simulink model "model_5LinkWalking"  (R2022b)
settings: Solver=ode45  StartTime=0.0  StopTime=Tf  FixedStep=1e-5  MaxStep=1e-3  RelTol=1e-12  AbsTol=1e-8
values from neighbouring files (symbols this model uses):
  f_dist = [0; -100; 0]    [main.m]    (also in main_5linkWalking_PSO.m)
  gains = [ ... (first row only)    [main.m]    (also in main_5linkWalking_PSO.m = [gain.kP1, gain.kD1, gain.kP2, gain.kD2, gain.kP3, gain.kD3,)
  gains_VSLIPSL = [gain_VSLIPSL.K_p; gain_VSLIPSL.K_d; gain_VSLIPSL.K_p_sw; gain_VSLIPSL.K_d_sw; gain_VSLIPSL.K_p_ds; gain_VSLIPSL.K_d_ds; gain_VSLIPSL.K_v_ds]    [main.m]    (also in main_5linkWalking_PSO.m)
  init_flag = [1; 0; -dc.col_param.footPlus; -slipsl.time_ss(N); slipsl.x_ss(1); slipsl.y_ss(1); alpha_ss_ref(1)]    [main.m]    (also in main_5linkWalking_PSO.m = [1; 0; -dc.col_param.footPlus; 0; CoM(1); CoM(2)])
  Initial_state = [q0;dq0]    [main.m]    (also in main_5linkWalking_PSO.m)
  param = [params.m1; params.m2; params.m5; params.l1; params.l2; params.l5; params.g; params.I1; params.I2; params.I5; params.r_k; params.r_h; params.k_ba; params.phi_h0; params.phi_k0]    [main.m]    (also in main_5linkWalking_PSO.m = [params.m1; params.m2; params.m5; params.l1; params.l2; para)
  ref_star_ds = [ref_star.ds.x_CoM_star,      ref_star.ds.y_CoM_star, ref_star.ds.dx_CoM_star,      ref_star.ds.del_y_CoM_star, ref_star.ds.del_dx_CoM_star,      ref_star.ds.del2_y_CoM_star]    [main.m]    (also in main_5linkWalking_PSO.m)
  ref_star_ss = [ref_star.ss.x_M_star,      ref_star.ss.y_M_star, ref_star.ss.x_swFoot_star, ref_star.ss.y_swFoot_star,      ref_star.ss.del_y_M_star, ref_star.ss.del_x_swFoot_star, ref_star.ss.del_y_swFoot_star,      ref_star.ss.del2_y_M_star, ref_star.ss.del2_x_swFoot_star, ref_star.ss.del2_y_swFoot_star,      ref_star.ss.x_CoM_star]    [main.m]    (also in main_5linkWalking_PSO.m)
  sample_time = 0.001    [main.m]    (also in main_5linkWalking_PSO.m)
  slipslParams = [ ... (first row only)    [main.m]    (also in main_5linkWalking_PSO.m)
  slipslTraj_ds = [slipsl.time_ds, slipsl.x_ds, slipsl.y_ds, slipsl.dx_ds, slipsl.dy_ds, alpha_ds_ref_discrete]    [main.m]    (also in main_5linkWalking_PSO.m = [ref_star.dc.ds.time - ref_star.dc.ds.time(1), ref_star.dc.d)
  slipslTraj_ss = [slipsl.time_ss, slipsl.x_ss, slipsl.y_ss, slipsl.dx_ss, slipsl.dy_ss, alpha_ss_ref_discrete]    [main.m]    (also in main_5linkWalking_PSO.m = [ref_star.dc.ss.time, ref_star.dc.ss.x_CoM', ref_star.dc.ss.)
  swFootTraj = [swFootSLIPSL.x_CoM, swFootSLIPSL.x, swFootSLIPSL.z, swFootSLIPSL.dx, swFootSLIPSL.dz]    [main.m]    (also in main_5linkWalking_PSO.m = [ref_star.dc.ss.x_CoM', ref_star.dc.ss.x_sw', ref_star.dc.ss)
libraries: simulink x1
(part 2 of 3)

== matlab function model_5LinkWalking/SLIP-SL Controller/SLIP-SL ==
  data: t input; des_traj output; X input; param input; flag input; slipslParams input; slipslTraj_ss input; slipslTraj_ds input; flag_des output; swFootTraj input; gains_VSLIPSL input; ref_star_ss input; ref_star_ds input; input_varStiff output; det_A_ds output; sw_ft_des output; des_th output; decoder_time_elapsed output; encoder_time_elapsed output
function [des_traj, flag_des, input_varStiff, det_A_ds, sw_ft_des, des_th, decoder_time_elapsed, encoder_time_elapsed] = fcn(t, X, param, flag, slipslParams, slipslTraj_ss, slipslTraj_ds, swFootTraj, gains_VSLIPSL, ref_star_ss, ref_star_ds)

%% variables (absolute angles)
th1 = X(1);
th2 = X(1) + X(2);
th3 = X(1) + X(2) + X(3);
th4 = X(1) + X(2) + X(3) + X(4);
th5 = X(1) + X(2) + X(5);

dth1 = X(6);
dth2 = X(6) + X(7);
dth3 = X(6) + X(7) + X(8);
dth4 = X(6) + X(7) + X(8) + X(9);
dth5 = X(6) + X(7) + X(10);

q = [th1;th2;th3;th4;th5];
dq = [dth1;dth2;dth3;dth4;dth5];

%% Parameters

m1 = param(1);
m2 = param(2);
m3 = m2;
m4 = m1;
m5 = param(3);

l1 = param(4);
l2 = param(5);
l5 = param(6);
l3 = l2;
l4 = l1;

gravi = param(7);
I1 = param(8);
I2 = param(9);
I5 = param(10);
I3 = I1;
I4 = I2;

%% flags
f_SS = flag(1); % indicates which stance phase it is
foot = flag(2); % location of the stance foot
foot_prev = flag(3); % previous location of the stance foot

t_mode_change = flag(4); % time stamp when the mode change happens (TD or LO)

x_LO = flag(5); % lift off location of CoM when it happened

%% CoM desired position and velocity calculation

time_ss = slipslTraj_ss(:,1);
x_slip_ss = slipslTraj_ss(:,2);
y_slip_ss = slipslTraj_ss(:,3);
dx_slip_ss = slipslTraj_ss(:,4);
dy_slip_ss = slipslTraj_ss(:,5);

time_ds = slipslTraj_ds(:,1);
x_slip_ds = slipslTraj_ds(:,2);
y_slip_ds = slipslTraj_ds(:,3);
dx_slip_ds = slipslTraj_ds(:,4);
dy_slip_ds = slipslTraj_ds(:,5);

CoM = calculate_com(X, param, foot, [0;0;0;0;0]); % calculating the location of CoM

x_CoM = CoM(1);
% z_CoM = CoM(2);
% dx_CoM = CoM(3); % velocity of CoM in x dir
% dz_CoM = CoM(4); % velocity of CoM in z dir

t_curr_step = t - t_mode_change; % timer for the current step, relative to the LO or TD time

if f_SS == 1
    % if we are in the SS phase
    
    if t_curr_step <= time_ss(end)
        % if the current time is within the SLIP-SL SS time
        
        x_CoM_des = interp1(time_ss, x_slip_ss, t_curr_step) + foot;
        y_CoM_des = interp1(time_ss, y_slip_ss, t_curr_step);
        dx_CoM_des = interp1(time_ss, dx_slip_ss, t_curr_step);
        dy_CoM_des = interp1(time_ss, dy_slip_ss, t_curr_step);
        
        flag_des = 1; % desired stance of the robot according to the slip traj
    else
        % if the current time has passed the time defined in SLIP-SL traj
        % (i.e. transition to DS is late)
        
%         x_CoM_des = x_slip_ss(end) + foot;
%         y_CoM_des = y_slip_ss(end);
%         dx_CoM_des = dx_slip_ss(end);
%         dy_CoM_des = dy_slip_ss(end);
        
        x_CoM_des = x_CoM; % current position of the x_CoM
        y_CoM_des = y_slip_ss(end);
        dx_CoM_des = dx_slip_ss(end);
        dy_CoM_des = dy_slip_ss(end);
        
        flag_des = 2; % desired stance of the robot according to the slip traj
    end
    
else
    % if we are in the DS phase
    
    footPlus = slipslParams(17); % position of footPlus for reference traj
    
    if t_curr_step <= time_ds(end)
        % if the current time is within the SLIP-SL DS time
        
        x_CoM_des = interp1(time_ds, x_slip_ds, t_curr_step) + foot - footPlus;
        y_CoM_des = interp1(time_ds, y_slip_ds, t_curr_step);
        dx_CoM_des = interp1(time_ds, dx_slip_ds, t_curr_step);
        dy_CoM_des = interp1(time_ds, dy_slip_ds, t_curr_step);
        
        flag_des = 2; % desired stance of the robot according to the slip traj
    else
        % if the current time has passed the time defined in SLIP-SL traj
        % (i.e. transition to SS is late)

        x_CoM_des = x_slip_ds(end) + foot - footPlus;
        y_CoM_des = y_slip_ds(end);
        dx_CoM_des = dx_slip_ds(end);
        dy_CoM_des = dy_slip_ds(end);
        
        flag_des = 1; % desired stance of the robot according to the slip traj
    end
end

%% SW foot desired position and velocity calculation

if f_SS == 1
    
    if t_curr_step <= time_ss(end)
        % if the x_CoM is within known SLIP-SL bounds
        x_sw_des = interp1(time_ss, swFootTraj(:,2) + foot, t_curr_step);
        y_sw_des = interp1(time_ss, swFootTraj(:,3), t_curr_step);
        dx_sw_des = interp1(time_ss, swFootTraj(:,4), t_curr_step);
        dy_sw_des = interp1(time_ss, swFootTraj(:,5), t_curr_step);
    else
        % if x_CoM goes out of SLIP-SL bounds, just use the last know ref. traj
        x_sw_des = swFootTraj(end,2) + foot;
        y_sw_des = swFootTraj(end,3);
        dx_sw_des = swFootTraj(end,4);
        % dy_sw_des = swFootTraj(end,5);
        dy_sw_des = swFootTraj(end,5) - 0.5*(t_curr_step - time_ss(end));
    end
    
else
    x_sw_des = foot_prev;
    y_sw_des = 0;
    dx_sw_des = 0;
    dy_sw_des = 0;
    
end

sw_ft_des = [x_sw_des; y_sw_des; dx_sw_des; dy_sw_des];

%% Desired accelerations calculation

% SLIP-SL constant params
m_M = slipslParams(1);
m_swLeg = slipslParams(2);
m_swFoot = slipslParams(3);
L_thigh = slipslParams(4);
I_swLeg = slipslParams(5);
I_swFoot = slipslParams(6);
gravi = slipslParams(7);

% SLIP-SL collocation parameters
k0_ss = slipslParams(8);
L0_ss = slipslParams(9);
k0_ds = slipslParams(10);
L0_ds = slipslParams(11);
k_swFoot = slipslParams(12);
k_swLeg = slipslParams(13);
theta0 = slipslParams(14);
r0 = slipslParams(15);
foot = slipslParams(16);
footPlus = slipslParams(17);

%%%%% V-SLIP-SL controller that calculates variable stiffness inputs %%%%%

% SS inputs
u1 = 0; % input for stance leg spring
u2 = 0; % input for swing leg torsional spring
u3 = 0; % input for swing foot spring
% DS inputs
u4 = 0; % input for stance leg spring
u5 = 0; % input for swing leg spring

% Controller Gains
K_p = gains_VSLIPSL(1);
K_d = gains_VSLIPSL(2);

K_p_sw = gains_VSLIPSL(3);
K_d_sw = gains_VSLIPSL(4);

K_p_ds = gains_VSLIPSL(5);
K_d_ds = gains_VSLIPSL(6);
K_v_ds = gains_VSLIPSL(7); % 5 in visser 2012

% for debugging
ref_output_ss = [0; 0; 0];
ref_output_ds = [0;0];
det_A_ss = -1;
det_A_ds = 0;

x_CoM_star_ds = ref_star_ds(:,1);
%%%%%%%%%%%%%%%%%%%%%%%%%%%%%%%%%%%%%%%%%%%%%%%%%%%%%%%%%%%%%%%%%%%%%%%%%%

encoder_time_elapsed = NaN;

if f_SS == 1
    % if the 5 link model is in SS
    
    if t_curr_step <= time_ss(end)
        % (SS) SLIP-SL states corresponding to current x_CoM position
        
        [x_M, y_M, theta, r, dx_M, dy_M, dtheta, dr, encoder_time_elapsed] = calc_5linkTOslipsl(X, flag, param, slipslParams);
        
        %%%%%% V-SLIP-SL SS Phase Controller %%%%%%%%%%%%%%%%%%%%%%%%%%%%%
        x_CoM_star_ss = ref_star_ss(:,11);
        x_M_star_ss = ref_star_ss(:,1);
        x_swFoot_ref = ref_star_ss(:,3);
        
        % updating the x_CoM_star_ss
        x_CoM_des_TD = ref_star_ss(end,11);
        x_CoM_star_ss = x_CoM_star_ss.*((x_CoM_des_TD - (x_LO-flag(2)))/(ref_star_ss(end,11) - ref_star_ss(1,11))) + ((x_LO-flag(2)) - ref_star_ss(1,11))/2;
        
        % calculating x_CoM when for SS phase
        x_swLeg = x_M + (L_thigh/2)*cos(theta);
        x_swFoot = x_M + (L_thigh + r)*cos(theta);
%         x_CoM = (m_M*x_M + m_swLeg*x_swLeg + m_swFoot*x_swFoot)/(m_M + m_swLeg + m_swFoot);
        x_CoM = CoM(1) - flag(2);
        
        if x_CoM_star_ss(1) <= x_CoM && x_CoM <= x_CoM_star_ss(end)
            %
            %     if x_M <= x_M_star_ss(end)
            
            % interpolation for references
            y_M_star = interp1(x_CoM_star_ss, ref_star_ss(:,2), x_CoM);
            %         x_swFoot_star = interp1(x_M_star_ss, x_swFoot_ref_mod, x_M);
            x_swFoot_star = interp1(x_CoM_star_ss, ref_star_ss(:,3), x_CoM);
            y_swFoot_star = interp1(x_CoM_star_ss, ref_star_ss(:,4), x_CoM);
            
            del_y_M_star = interp1(x_CoM_star_ss, ref_star_ss(:,5), x_CoM);
            del_x_swFoot_star = interp1(x_CoM_star_ss, ref_star_ss(:,6), x_CoM);
            del_y_swFoot_star = interp1(x_CoM_star_ss, ref_star_ss(:,7), x_CoM);
            
            del2_y_M_star = interp1(x_CoM_star_ss, ref_star_ss(:,8), x_CoM);
            del2_x_swFoot_star = interp1(x_CoM_star_ss, ref_star_ss(:,9), x_CoM);
            del2_y_swFoot_star = interp1(x_CoM_star_ss, ref_star_ss(:,10), x_CoM);

%             % interpolation for references (trying time based instead of x_CoM based
%             y_M_star = interp1(x_CoM_star_ss, ref_star_ss(:,2), x_CoM);
%             %         x_swFoot_star = interp1(x_M_star_ss, x_swFoot_ref_mod, x_M);
%             x_swFoot_star = interp1(x_CoM_star_ss, ref_star_ss(:,3), x_CoM);
%             y_swFoot_star = interp1(x_CoM_star_ss, ref_star_ss(:,4), x_CoM);
%             
%             del_y_M_star = interp1(x_CoM_star_ss, ref_star_ss(:,5), x_CoM);
%             del_x_swFoot_star = interp1(x_CoM_star_ss, ref_star_ss(:,6), x_CoM);
%             del_y_swFoot_star = interp1(x_CoM_star_ss, ref_star_ss(:,7), x_CoM);
%             
%             del2_y_M_star = interp1(x_CoM_star_ss, ref_star_ss(:,8), x_CoM);
%             del2_x_swFoot_star = interp1(x_CoM_star_ss, ref_star_ss(:,9), x_CoM);
%             del2_y_swFoot_star = interp1(x_CoM_star_ss, ref_star_ss(:,10), x_CoM);
            
            ref_output_ss = [y_M_star; x_swFoot_star; y_swFoot_star];
            
            % controller
            
            A_ss = [
                ((L0_ss - (x_M^2 + y_M^2)^(1/2))*(L_thigh^2*m_swLeg^2*y_M + 8*I_swLeg*m_M*y_M + 8*I_swFoot*m_M*y_M + 8*I_swLeg*m_swLeg*y_M + 4*I_swLeg*m_swFoot*y_M + 8*I_swFoot*m_swLeg*y_M + 4*I_swFoot*m_swFoot*y_M + 2*L_thigh^2*m_M*m_swLeg*y_M + 8*L_thigh^2*m_M*m_swFoot*y_M + 5*L_thigh^2*m_swLeg*m_swFoot*y_M + 8*m_M*m_swFoot*r^2*y_M + 8*m_swLeg*m_swFoot*r^2*y_M + L_thigh^2*m_swLeg^2*y_M*cos(2*theta) - L_thigh^2*m_swLeg^2*x_M*sin(2*theta) - 4*I_swLeg*m_swFoot*y_M*cos(2*theta) - 4*I_swFoot*m_swFoot*y_M*cos(2*theta) + 4*I_swLeg*m_swFoot*x_M*sin(2*theta) + 4*I_swFoot*m_swFoot*x_M*sin(2*theta) + 16*L_thigh*m_M*m_swFoot*r*y_M + 12*L_thigh*m_swLeg*m_swFoot*r*y_M + 3*L_thigh^2*m_swLeg*m_swFoot*y_M*cos(2*theta) - 3*L_thigh^2*m_swLeg*m_swFoot*x_M*sin(2*theta) + 4*L_thigh*m_swLeg*m_swFoot*r*y_M*cos(2*theta) - 4*L_thigh*m_swLeg*m_swFoot*r*x_M*sin(2*theta)))/(2*(x_M^2 + y_M^2)^(1/2)*(m_M + m_swLeg)*(4*I_swLeg*m_M + 4*I_swFoot*m_M + 4*I_swLeg*m_swLeg + 4*I_swLeg*m_swFoot + 4*I_swFoot*m_swLeg + 4*I_swFoot*m_swFoot + 4*m_M*m_swFoot*r^2 + 4*m_swLeg*m_swFoot*r^2 + L_thigh^2*m_M*m_swLeg + 4*L_thigh^2*m_M*m_swFoot + L_thigh^2*m_swLeg*m_swFoot + 8*L_thigh*m_M*m_swFoot*r + 4*L_thigh*m_swLeg*m_swFoot*r)) - (del_y_M_star*(L0_ss - (x_M^2 + y_M^2)^(1/2))*((L_thigh^2*m_swLeg^2*x_M)/2 + 4*I_swLeg*m_M*x_M + 4*I_swFoot*m_M*x_M + 4*I_swLeg*m_swLeg*x_M + 2*I_swLeg*m_swFoot*x_M + 4*I_swFoot*m_swLeg*x_M + 2*I_swFoot*m_swFoot*x_M + L_thigh^2*m_M*m_swLeg*x_M + 4*L_thigh^2*m_M*m_swFoot*x_M + (5*L_thigh^2*m_swLeg*m_swFoot*x_M)/2 + 4*m_M*m_swFoot*r^2*x_M + 4*m_swLeg*m_swFoot*r^2*x_M - (L_thigh^2*m_swLeg^2*x_M*cos(2*theta))/2 - (L_thigh^2*m_swLeg^2*y_M*sin(2*theta))/2 + 2*I_swLeg*m_swFoot*x_M*cos(2*theta) + 2*I_swFoot*m_swFoot*x_M*cos(2*theta) + 2*I_swLeg*m_swFoot*y_M*sin(2*theta) + 2*I_swFoot*m_swFoot*y_M*sin(2*theta) + 8*L_thigh*m_M*m_swFoot*r*x_M + 6*L_thigh*m_swLeg*m_swFoot*r*x_M - (3*L_thigh^2*m_swLeg*m_swFoot*x_M*cos(2*theta))/2 - (3*L_thigh^2*m_swLeg*m_swFoot*y_M*sin(2*theta))/2 - 2*L_thigh*m_swLeg*m_swFoot*r*x_M*cos(2*theta) - 2*L_thigh*m_swLeg*m_swFoot*r*y_M*sin(2*theta)))/((x_M^2 + y_M^2)^(1/2)*(m_M + m_swLeg)*(4*I_swLeg*m_M + 4*I_swFoot*m_M + 4*I_swLeg*m_swLeg + 4*I_swLeg*m_swFoot + 4*I_swFoot*m_swLeg + 4*I_swFoot*m_swFoot + 4*m_M*m_swFoot*r^2 + 4*m_swLeg*m_swFoot*r^2 + L_thigh^2*m_M*m_swLeg + 4*L_thigh^2*m_M*m_swFoot + L_thigh^2*m_swLeg*m_swFoot + 8*L_thigh*m_M*m_swFoot*r + 4*L_thigh*m_swLeg*m_swFoot*r)),                                                                                                                                                        (2*(theta - theta0)*(cos(theta) + del_y_M_star*sin(theta))*(L_thigh*m_swLeg + 2*L_thigh*m_swFoot + 2*m_swFoot*r))/(4*I_swLeg*m_M + 4*I_swFoot*m_M + 4*I_swLeg*m_swLeg + 4*I_swLeg*m_swFoot + 4*I_swFoot*m_swLeg + 4*I_swFoot*m_swFoot + 4*m_M*m_swFoot*r^2 + 4*m_swLeg*m_swFoot*r^2 + L_thigh^2*m_M*m_swLeg + 4*L_thigh^2*m_M*m_swFoot + L_thigh^2*m_swLeg*m_swFoot + 8*L_thigh*m_M*m_swFoot*r + 4*L_thigh*m_swLeg*m_swFoot*r),                                                    ((r - r0)*(sin(theta) - del_y_M_star*cos(theta)))/(m_M + m_swLeg)
                (2*sin(theta)*(L_thigh + r)*(L0_ss - (x_M^2 + y_M^2)^(1/2))*(y_M*cos(theta) - x_M*sin(theta))*(L_thigh*m_swLeg + 2*L_thigh*m_swFoot + 2*m_swFoot*r))/((x_M^2 + y_M^2)^(1/2)*(4*I_swLeg*m_M + 4*I_swFoot*m_M + 4*I_swLeg*m_swLeg + 4*I_swLeg*m_swFoot + 4*I_swFoot*m_swLeg + 4*I_swFoot*m_swFoot + 4*m_M*m_swFoot*r^2 + 4*m_swLeg*m_swFoot*r^2 + L_thigh^2*m_M*m_swLeg + 4*L_thigh^2*m_M*m_swFoot + L_thigh^2*m_swLeg*m_swFoot + 8*L_thigh*m_M*m_swFoot*r + 4*L_thigh*m_swLeg*m_swFoot*r)) - ((L0_ss - (x_M^2 + y_M^2)^(1/2))*(del_x_swFoot_star - 1)*((L_thigh^2*m_swLeg^2*x_M)/2 + 4*I_swLeg*m_M*x_M + 4*I_swFoot*m_M*x_M + 4*I_swLeg*m_swLeg*x_M + 2*I_swLeg*m_swFoot*x_M + 4*I_swFoot*m_swLeg*x_M + 2*I_swFoot*m_swFoot*x_M + L_thigh^2*m_M*m_swLeg*x_M + 4*L_thigh^2*m_M*m_swFoot*x_M + (5*L_thigh^2*m_swLeg*m_swFoot*x_M)/2 + 4*m_M*m_swFoot*r^2*x_M + 4*m_swLeg*m_swFoot*r^2*x_M - (L_thigh^2*m_swLeg^2*x_M*cos(2*theta))/2 - (L_thigh^2*m_swLeg^2*y_M*sin(2*theta))/2 + 2*I_swLeg*m_swFoot*x_M*cos(2*theta) + 2*I_swFoot*m_swFoot*x_M*cos(2*theta) + 2*I_swLeg*m_swFoot*y_M*sin(2*theta) + 2*I_swFoot*m_swFoot*y_M*sin(2*theta) + 8*L_thigh*m_M*m_swFoot*r*x_M + 6*L_thigh*m_swLeg*m_swFoot*r*x_M - (3*L_thigh^2*m_swLeg*m_swFoot*x_M*cos(2*theta))/2 - (3*L_thigh^2*m_swLeg*m_swFoot*y_M*sin(2*theta))/2 - 2*L_thigh*m_swLeg*m_swFoot*r*x_M*cos(2*theta) - 2*L_thigh*m_swLeg*m_swFoot*r*y_M*sin(2*theta)))/((x_M^2 + y_M^2)^(1/2)*(m_M + m_swLeg)*(4*I_swLeg*m_M + 4*I_swFoot*m_M + 4*I_swLeg*m_swLeg + 4*I_swLeg*m_swFoot + 4*I_swFoot*m_swLeg + 4*I_swFoot*m_swFoot + 4*m_M*m_swFoot*r^2 + 4*m_swLeg*m_swFoot*r^2 + L_thigh^2*m_M*m_swLeg + 4*L_thigh^2*m_M*m_swFoot + L_thigh^2*m_swLeg*m_swFoot + 8*L_thigh*m_M*m_swFoot*r + 4*L_thigh*m_swLeg*m_swFoot*r)) - (cos(theta)*(L0_ss - (x_M^2 + y_M^2)^(1/2))*(x_M*cos(theta) + y_M*sin(theta)))/((x_M^2 + y_M^2)^(1/2)*(m_M + m_swLeg)),                                                                    (2*sin(theta)*(theta - theta0)*(2*L_thigh*m_M + L_thigh*m_swLeg + 2*m_M*r + 2*m_swLeg*r + L_thigh*del_x_swFoot_star*m_swLeg + 2*L_thigh*del_x_swFoot_star*m_swFoot + 2*del_x_swFoot_star*m_swFoot*r))/(4*I_swLeg*m_M + 4*I_swFoot*m_M + 4*I_swLeg*m_swLeg + 4*I_swLeg*m_swFoot + 4*I_swFoot*m_swLeg + 4*I_swFoot*m_swFoot + 4*m_M*m_swFoot*r^2 + 4*m_swLeg*m_swFoot*r^2 + L_thigh^2*m_M*m_swLeg + 4*L_thigh^2*m_M*m_swFoot + L_thigh^2*m_swLeg*m_swFoot + 8*L_thigh*m_M*m_swFoot*r + 4*L_thigh*m_swLeg*m_swFoot*r),                       -(cos(theta)*(r - r0)*(m_M + m_swLeg + del_x_swFoot_star*m_swFoot))/(m_swFoot*(m_M + m_swLeg))
                ((L0_ss - (x_M^2 + y_M^2)^(1/2))*(L_thigh^2*m_swLeg^2*y_M + 8*I_swLeg*m_M*y_M + 8*I_swFoot*m_M*y_M + 8*I_swLeg*m_swLeg*y_M + 4*I_swLeg*m_swFoot*y_M + 8*I_swFoot*m_swLeg*y_M + 4*I_swFoot*m_swFoot*y_M + 2*L_thigh^2*m_M*m_swLeg*y_M + 8*L_thigh^2*m_M*m_swFoot*y_M + 5*L_thigh^2*m_swLeg*m_swFoot*y_M + 8*m_M*m_swFoot*r^2*y_M + 8*m_swLeg*m_swFoot*r^2*y_M + L_thigh^2*m_swLeg^2*y_M*cos(2*theta) - L_thigh^2*m_swLeg^2*x_M*sin(2*theta) - 4*I_swLeg*m_swFoot*y_M*cos(2*theta) - 4*I_swFoot*m_swFoot*y_M*cos(2*theta) + 4*I_swLeg*m_swFoot*x_M*sin(2*theta) + 4*I_swFoot*m_swFoot*x_M*sin(2*theta) + 16*L_thigh*m_M*m_swFoot*r*y_M + 12*L_thigh*m_swLeg*m_swFoot*r*y_M + 3*L_thigh^2*m_swLeg*m_swFoot*y_M*cos(2*theta) - 3*L_thigh^2*m_swLeg*m_swFoot*x_M*sin(2*theta) + 4*L_thigh*m_swLeg*m_swFoot*r*y_M*cos(2*theta) - 4*L_thigh*m_swLeg*m_swFoot*r*x_M*sin(2*theta)))/(2*(x_M^2 + y_M^2)^(1/2)*(m_M + m_swLeg)*(4*I_swLeg*m_M + 4*I_swFoot*m_M + 4*I_swLeg*m_swLeg + 4*I_swLeg*m_swFoot + 4*I_swFoot*m_swLeg + 4*I_swFoot*m_swFoot + 4*m_M*m_swFoot*r^2 + 4*m_swLeg*m_swFoot*r^2 + L_thigh^2*m_M*m_swLeg + 4*L_thigh^2*m_M*m_swFoot + L_thigh^2*m_swLeg*m_swFoot + 8*L_thigh*m_M*m_swFoot*r + 4*L_thigh*m_swLeg*m_swFoot*r)) - (sin(theta)*(L0_ss - (x_M^2 + y_M^2)^(1/2))*(x_M*cos(theta) + y_M*sin(theta)))/((x_M^2 + y_M^2)^(1/2)*(m_M + m_swLeg)) - (del_y_swFoot_star*(L0_ss - (x_M^2 + y_M^2)^(1/2))*((L_thigh^2*m_swLeg^2*x_M)/2 + 4*I_swLeg*m_M*x_M + 4*I_swFoot*m_M*x_M + 4*I_swLeg*m_swLeg*x_M + 2*I_swLeg*m_swFoot*x_M + 4*I_swFoot*m_swLeg*x_M + 2*I_swFoot*m_swFoot*x_M + L_thigh^2*m_M*m_swLeg*x_M + 4*L_thigh^2*m_M*m_swFoot*x_M + (5*L_thigh^2*m_swLeg*m_swFoot*x_M)/2 + 4*m_M*m_swFoot*r^2*x_M + 4*m_swLeg*m_swFoot*r^2*x_M - (L_thigh^2*m_swLeg^2*x_M*cos(2*theta))/2 - (L_thigh^2*m_swLeg^2*y_M*sin(2*theta))/2 + 2*I_swLeg*m_swFoot*x_M*cos(2*theta) + 2*I_swFoot*m_swFoot*x_M*cos(2*theta) + 2*I_swLeg*m_swFoot*y_M*sin(2*theta) + 2*I_swFoot*m_swFoot*y_M*sin(2*theta) + 8*L_thigh*m_M*m_swFoot*r*x_M + 6*L_thigh*m_swLeg*m_swFoot*r*x_M - (3*L_thigh^2*m_swLeg*m_swFoot*x_M*cos(2*theta))/2 - (3*L_thigh^2*m_swLeg*m_swFoot*y_M*sin(2*theta))/2 - 2*L_thigh*m_swLeg*m_swFoot*r*x_M*cos(2*theta) - 2*L_thigh*m_swLeg*m_swFoot*r*y_M*sin(2*theta)))/((x_M^2 + y_M^2)^(1/2)*(m_M + m_swLeg)*(4*I_swLeg*m_M + 4*I_swFoot*m_M + 4*I_swLeg*m_swLeg + 4*I_swLeg*m_swFoot + 4*I_swFoot*m_swLeg + 4*I_swFoot*m_swFoot + 4*m_M*m_swFoot*r^2 + 4*m_swLeg*m_swFoot*r^2 + L_thigh^2*m_M*m_swLeg + 4*L_thigh^2*m_M*m_swFoot + L_thigh^2*m_swLeg*m_swFoot + 8*L_thigh*m_M*m_swFoot*r + 4*L_thigh*m_swLeg*m_swFoot*r)) - (2*cos(theta)*(L_thigh + r)*(L0_ss - (x_M^2 + y_M^2)^(1/2))*(y_M*cos(theta) - x_M*sin(theta))*(L_thigh*m_swLeg + 2*L_thigh*m_swFoot + 2*m_swFoot*r))/((x_M^2 + y_M^2)^(1/2)*(4*I_swLeg*m_M + 4*I_swFoot*m_M + 4*I_swLeg*m_swLeg + 4*I_swLeg*m_swFoot + 4*I_swFoot*m_swLeg + 4*I_swFoot*m_swFoot + 4*m_M*m_swFoot*r^2 + 4*m_swLeg*m_swFoot*r^2 + L_thigh^2*m_M*m_swLeg + 4*L_thigh^2*m_M*m_swFoot + L_thigh^2*m_swLeg*m_swFoot + 8*L_thigh*m_M*m_swFoot*r + 4*L_thigh*m_swLeg*m_swFoot*r)), -(2*(theta - theta0)*(2*m_M*r*cos(theta) + 2*m_swLeg*r*cos(theta) + 2*L_thigh*m_M*cos(theta) + L_thigh*m_swLeg*cos(theta) - L_thigh*del_y_swFoot_star*m_swLeg*sin(theta) - 2*L_thigh*del_y_swFoot_star*m_swFoot*sin(theta) - 2*del_y_swFoot_star*m_swFoot*r*sin(theta)))/(4*I_swLeg*m_M + 4*I_swFoot*m_M + 4*I_swLeg*m_swLeg + 4*I_swLeg*m_swFoot + 4*I_swFoot*m_swLeg + 4*I_swFoot*m_swFoot + 4*m_M*m_swFoot*r^2 + 4*m_swLeg*m_swFoot*r^2 + L_thigh^2*m_M*m_swLeg + 4*L_thigh^2*m_M*m_swFoot + L_thigh^2*m_swLeg*m_swFoot + 8*L_thigh*m_M*m_swFoot*r + 4*L_thigh*m_swLeg*m_swFoot*r), -((r - r0)*(m_M*sin(theta) + m_swLeg*sin(theta) + del_y_swFoot_star*m_swFoot*cos(theta)))/(m_swFoot*(m_M + m_swLeg))];
            
            K_ss = [
                del2_y_M_star*dx_M^2 - K_p*(y_M - y_M_star) - K_d*(dy_M - del_y_M_star*dx_M) + (8*I_swLeg*gravi*m_M^2*(x_M^2 + y_M^2)^(1/2) + 8*I_swFoot*gravi*m_M^2*(x_M^2 + y_M^2)^(1/2) + 8*I_swLeg*gravi*m_swLeg^2*(x_M^2 + y_M^2)^(1/2) + 8*I_swFoot*gravi*m_swLeg^2*(x_M^2 + y_M^2)^(1/2) - L0_ss*L_thigh^2*k0_ss*m_swLeg^2*y_M + 2*L_thigh^2*gravi*m_M*m_swLeg^2*(x_M^2 + y_M^2)^(1/2) + 2*L_thigh^2*gravi*m_M^2*m_swLeg*(x_M^2 + y_M^2)^(1/2) + 8*L_thigh^2*gravi*m_M^2*m_swFoot*(x_M^2 + y_M^2)^(1/2) + 2*L_thigh^2*gravi*m_swLeg^2*m_swFoot*(x_M^2 + y_M^2)^(1/2) + L_thigh^2*k0_ss*m_swLeg^2*y_M*(x_M^2 + y_M^2)^(1/2) + 8*gravi*m_M^2*m_swFoot*r^2*(x_M^2 + y_M^2)^(1/2) + 8*gravi*m_swLeg^2*m_swFoot*r^2*(x_M^2 + y_M^2)^(1/2) - 8*I_swLeg*L0_ss*k0_ss*m_M*y_M - 8*I_swFoot*L0_ss*k0_ss*m_M*y_M - 8*I_swLeg*L0_ss*k0_ss*m_swLeg*y_M - 4*I_swLeg*L0_ss*k0_ss*m_swFoot*y_M - 8*I_swFoot*L0_ss*k0_ss*m_swLeg*y_M - 4*I_swFoot*L0_ss*k0_ss*m_swFoot*y_M + 16*I_swLeg*gravi*m_M*m_swLeg*(x_M^2 + y_M^2)^(1/2) + 8*I_swLeg*gravi*m_M*m_swFoot*(x_M^2 + y_M^2)^(1/2) + 16*I_swFoot*gravi*m_M*m_swLeg*(x_M^2 + y_M^2)^(1/2) + 8*I_swFoot*gravi*m_M*m_swFoot*(x_M^2 + y_M^2)^(1/2) + 8*I_swLeg*gravi*m_swLeg*m_swFoot*(x_M^2 + y_M^2)^(1/2) + 8*I_swFoot*gravi*m_swLeg*m_swFoot*(x_M^2 + y_M^2)^(1/2) + 8*I_swLeg*k0_ss*m_M*y_M*(x_M^2 + y_M^2)^(1/2) + 8*I_swFoot*k0_ss*m_M*y_M*(x_M^2 + y_M^2)^(1/2) + 8*I_swLeg*k0_ss*m_swLeg*y_M*(x_M^2 + y_M^2)^(1/2) + 4*I_swLeg*k0_ss*m_swFoot*y_M*(x_M^2 + y_M^2)^(1/2) + 8*I_swFoot*k0_ss*m_swLeg*y_M*(x_M^2 + y_M^2)^(1/2) + 4*I_swFoot*k0_ss*m_swFoot*y_M*(x_M^2 + y_M^2)^(1/2) - 2*L0_ss*L_thigh^2*k0_ss*m_M*m_swLeg*y_M - 8*L0_ss*L_thigh^2*k0_ss*m_M*m_swFoot*y_M - 5*L0_ss*L_thigh^2*k0_ss*m_swLeg*m_swFoot*y_M + 10*L_thigh^2*gravi*m_M*m_swLeg*m_swFoot*(x_M^2 + y_M^2)^(1/2) + 16*L_thigh*gravi*m_M^2*m_swFoot*r*(x_M^2 + y_M^2)^(1/2) + 8*L_thigh*gravi*m_swLeg^2*m_swFoot*r*(x_M^2 + y_M^2)^(1/2) + 2*L_thigh^2*k0_ss*m_M*m_swLeg*y_M*(x_M^2 + y_M^2)^(1/2) + 8*L_thigh^2*k0_ss*m_M*m_swFoot*y_M*(x_M^2 + y_M^2)^(1/2) + 5*L_thigh^2*k0_ss*m_swLeg*m_swFoot*y_M*(x_M^2 + y_M^2)^(1/2) - 8*L0_ss*k0_ss*m_M*m_swFoot*r^2*y_M - 8*L0_ss*k0_ss*m_swLeg*m_swFoot*r^2*y_M - L0_ss*L_thigh^2*k0_ss*m_swLeg^2*y_M*cos(2*theta) - 8*I_swLeg*k_swFoot*m_M*r*sin(theta)*(x_M^2 + y_M^2)^(1/2) + 8*I_swLeg*k_swFoot*m_M*r0*sin(theta)*(x_M^2 + y_M^2)^(1/2) - 8*I_swFoot*k_swFoot*m_M*r*sin(theta)*(x_M^2 + y_M^2)^(1/2) + 8*I_swFoot*k_swFoot*m_M*r0*sin(theta)*(x_M^2 + y_M^2)^(1/2) - 8*I_swLeg*k_swFoot*m_swLeg*r*sin(theta)*(x_M^2 + y_M^2)^(1/2) + 8*I_swLeg*k_swFoot*m_swLeg*r0*sin(theta)*(x_M^2 + y_M^2)^(1/2) - 8*I_swLeg*k_swFoot*m_swFoot*r*sin(theta)*(x_M^2 + y_M^2)^(1/2) + 8*I_swLeg*k_swFoot*m_swFoot*r0*sin(theta)*(x_M^2 + y_M^2)^(1/2) - 8*I_swFoot*k_swFoot*m_swLeg*r*sin(theta)*(x_M^2 + y_M^2)^(1/2) + 8*I_swFoot*k_swFoot*m_swLeg*r0*sin(theta)*(x_M^2 + y_M^2)^(1/2) - 8*I_swFoot*k_swFoot*m_swFoot*r*sin(theta)*(x_M^2 + y_M^2)^(1/2) + 8*I_swFoot*k_swFoot*m_swFoot*r0*sin(theta)*(x_M^2 + y_M^2)^(1/2) + L0_ss*L_thigh^2*k0_ss*m_swLeg^2*x_M*sin(2*theta) + 16*gravi*m_M*m_swLeg*m_swFoot*r^2*(x_M^2 + y_M^2)^(1/2) + 8*k0_ss*m_M*m_swFoot*r^2*y_M*(x_M^2 + y_M^2)^(1/2) + 8*k0_ss*m_swLeg*m_swFoot*r^2*y_M*(x_M^2 + y_M^2)^(1/2) - L_thigh^3*dtheta^2*m_M*m_swLeg^2*sin(theta)*(x_M^2 + y_M^2)^(1/2) - L_thigh^3*dtheta^2*m_swLeg^2*m_swFoot*sin(theta)*(x_M^2 + y_M^2)^(1/2) + L_thigh^2*k0_ss*m_swLeg^2*y_M*cos(2*theta)*(x_M^2 + y_M^2)^(1/2) - L_thigh^2*k0_ss*m_swLeg^2*x_M*sin(2*theta)*(x_M^2 + y_M^2)^(1/2) + 4*I_swLeg*L0_ss*k0_ss*m_swFoot*y_M*cos(2*theta) + 4*I_swFoot*L0_ss*k0_ss*m_swFoot*y_M*cos(2*theta) - 4*I_swLeg*L0_ss*k0_ss*m_swFoot*x_M*sin(2*theta) - 4*I_swFoot*L0_ss*k0_ss*m_swFoot*x_M*sin(2*theta) - 4*L_thigh*k_swLeg*m_swLeg^2*theta*cos(theta)*(x_M^2 + y_M^2)^(1/2) + 4*L_thigh*k_swLeg*m_swLeg^2*theta0*cos(theta)*(x_M^2 + y_M^2)^(1/2) - 4*I_swLeg*k0_ss*m_swFoot*y_M*cos(2*theta)*(x_M^2 + y_M^2)^(1/2) - 4*I_swFoot*k0_ss*m_swFoot*y_M*cos(2*theta)*(x_M^2 + y_M^2)^(1/2) + 4*I_swLeg*k0_ss*m_swFoot*x_M*sin(2*theta)*(x_M^2 + y_M^2)^(1/2) + 4*I_swFoot*k0_ss*m_swFoot*x_M*sin(2*theta)*(x_M^2 + y_M^2)^(1/2) - 8*k_swFoot*m_M*m_swFoot*r^3*sin(theta)*(x_M^2 + y_M^2)^(1/2) - 8*k_swFoot*m_swLeg*m_swFoot*r^3*sin(theta)*(x_M^2 + y_M^2)^(1/2) - 4*I_swLeg*L_thigh*dtheta^2*m_swLeg^2*sin(theta)*(x_M^2 + y_M^2)^(1/2) - 4*I_swFoot*L_thigh*dtheta^2*m_swLeg^2*sin(theta)*(x_M^2 + y_M^2)^(1/2) - 2*L_thigh^2*k_swFoot*m_M*m_swLeg*r*sin(theta)*(x_M^2 + y_M^2)^(1/2) + 2*L_thigh^2*k_swFoot*m_M*m_swLeg*r0*sin(theta)*(x_M^2 + y_M^2)^(1/2) - 16*L_thigh*k_swFoot*m_M*m_swFoot*r^2*sin(theta)*(x_M^2 + y_M^2)^(1/2) - 8*L_thigh^2*k_swFoot*m_M*m_swFoot*r*sin(theta)*(x_M^2 + y_M^2)^(1/2) + 8*L_thigh^2*k_swFoot*m_M*m_swFoot*r0*sin(theta)*(x_M^2 + y_M^2)^(1/2) - 8*L_thigh*k_swFoot*m_swLeg*m_swFoot*r^2*sin(theta)*(x_M^2 + y_M^2)^(1/2) - 2*L_thigh^2*k_swFoot*m_swLeg*m_swFoot*r*sin(theta)*(x_M^2 + y_M^2)^(1/2) + 2*L_thigh^2*k_swFoot*m_swLeg*m_swFoot*r0*sin(theta)*(x_M^2 + y_M^2)^(1/2) - 16*L0_ss*L_thigh*k0_ss*m_M*m_swFoot*r*y_M - 12*L0_ss*L_thigh*k0_ss*m_swLeg*m_swFoot*r*y_M + 24*L_thigh*gravi*m_M*m_swLeg*m_swFoot*r*(x_M^2 + y_M^2)^(1/2) + 8*k_swFoot*m_M*m_swFoot*r^2*r0*sin(theta)*(x_M^2 + y_M^2)^(1/2) + 8*k_swFoot*m_swLeg*m_swFoot*r^2*r0*sin(theta)*(x_M^2 + y_M^2)^(1/2) + 16*L_thigh*k0_ss*m_M*m_swFoot*r*y_M*(x_M^2 + y_M^2)^(1/2) + 12*L_thigh*k0_ss*m_swLeg*m_swFoot*r*y_M*(x_M^2 + y_M^2)^(1/2) - 3*L0_ss*L_thigh^2*k0_ss*m_swLeg*m_swFoot*y_M*cos(2*theta) - 4*L_thigh^2*dr*dtheta*m_swLeg^2*m_swFoot*cos(theta)*(x_M^2 + y_M^2)^(1/2) + 3*L0_ss*L_thigh^2*k0_ss*m_swLeg*m_swFoot*x_M*sin(2*theta) - 4*L_thigh^3*dtheta^2*m_M*m_swLeg*m_swFoot*sin(theta)*(x_M^2 + y_M^2)^(1/2) + 3*L_thigh^2*k0_ss*m_swLeg*m_swFoot*y_M*cos(2*theta)*(x_M^2 + y_M^2)^(1/2) - 3*L_thigh^2*k0_ss*m_swLeg*m_swFoot*x_M*sin(2*theta)*(x_M^2 + y_M^2)^(1/2) + 16*I_swLeg*dr*dtheta*m_M*m_swFoot*cos(theta)*(x_M^2 + y_M^2)^(1/2) + 16*I_swFoot*dr*dtheta*m_M*m_swFoot*cos(theta)*(x_M^2 + y_M^2)^(1/2) + 16*I_swLeg*dr*dtheta*m_swLeg*m_swFoot*cos(theta)*(x_M^2 + y_M^2)^(1/2) + 16*I_swFoot*dr*dtheta*m_swLeg*m_swFoot*cos(theta)*(x_M^2 + y_M^2)^(1/2) - 4*L_thigh*k_swLeg*m_M*m_swLeg*theta*cos(theta)*(x_M^2 + y_M^2)^(1/2) + 4*L_thigh*k_swLeg*m_M*m_swLeg*theta0*cos(theta)*(x_M^2 + y_M^2)^(1/2) - 8*L_thigh*k_swLeg*m_M*m_swFoot*theta*cos(theta)*(x_M^2 + y_M^2)^(1/2) + 8*L_thigh*k_swLeg*m_M*m_swFoot*theta0*cos(theta)*(x_M^2 + y_M^2)^(1/2) - 8*L_thigh*k_swLeg*m_swLeg*m_swFoot*theta*cos(theta)*(x_M^2 + y_M^2)^(1/2) + 8*L_thigh*k_swLeg*m_swLeg*m_swFoot*theta0*cos(theta)*(x_M^2 + y_M^2)^(1/2) - 4*L_thigh*dtheta^2*m_swLeg^2*m_swFoot*r^2*sin(theta)*(x_M^2 + y_M^2)^(1/2) - 4*L_thigh^2*dtheta^2*m_swLeg^2*m_swFoot*r*sin(theta)*(x_M^2 + y_M^2)^(1/2) - 8*k_swLeg*m_M*m_swFoot*r*theta*cos(theta)*(x_M^2 + y_M^2)^(1/2) + 8*k_swLeg*m_M*m_swFoot*r*theta0*cos(theta)*(x_M^2 + y_M^2)^(1/2) - 8*k_swLeg*m_swLeg*m_swFoot*r*theta*cos(theta)*(x_M^2 + y_M^2)^(1/2) + 8*k_swLeg*m_swLeg*m_swFoot*r*theta0*cos(theta)*(x_M^2 + y_M^2)^(1/2) - 4*I_swLeg*L_thigh*dtheta^2*m_M*m_swLeg*sin(theta)*(x_M^2 + y_M^2)^(1/2) - 4*I_swFoot*L_thigh*dtheta^2*m_M*m_swLeg*sin(theta)*(x_M^2 + y_M^2)^(1/2) - 4*I_swLeg*L_thigh*dtheta^2*m_swLeg*m_swFoot*sin(theta)*(x_M^2 + y_M^2)^(1/2) - 4*I_swFoot*L_thigh*dtheta^2*m_swLeg*m_swFoot*sin(theta)*(x_M^2 + y_M^2)^(1/2) + 16*L_thigh*k_swFoot*m_M*m_swFoot*r*r0*sin(theta)*(x_M^2 + y_M^2)^(1/2) + 8*L_thigh*k_swFoot*m_swLeg*m_swFoot*r*r0*sin(theta)*(x_M^2 + y_M^2)^(1/2) - 4*L0_ss*L_thigh*k0_ss*m_swLeg*m_swFoot*r*y_M*cos(2*theta) - 4*L_thigh^2*dr*dtheta*m_M*m_swLeg*m_swFoot*cos(theta)*(x_M^2 + y_M^2)^(1/2) - 8*L_thigh*dr*dtheta*m_swLeg^2*m_swFoot*r*cos(theta)*(x_M^2 + y_M^2)^(1/2) + 4*L0_ss*L_thigh*k0_ss*m_swLeg*m_swFoot*r*x_M*sin(2*theta) + 4*L_thigh*k0_ss*m_swLeg*m_swFoot*r*y_M*cos(2*theta)*(x_M^2 + y_M^2)^(1/2) - 4*L_thigh*k0_ss*m_swLeg*m_swFoot*r*x_M*sin(2*theta)*(x_M^2 + y_M^2)^(1/2) - 4*L_thigh*dtheta^2*m_M*m_swLeg*m_swFoot*r^2*sin(theta)*(x_M^2 + y_M^2)^(1/2) - 8*L_thigh^2*dtheta^2*m_M*m_swLeg*m_swFoot*r*sin(theta)*(x_M^2 + y_M^2)^(1/2) - 8*L_thigh*dr*dtheta*m_M*m_swLeg*m_swFoot*r*cos(theta)*(x_M^2 + y_M^2)^(1/2))/(2*(x_M^2 + y_M^2)^(1/2)*(m_M + m_swLeg)*(4*I_swLeg*m_M + 4*I_swFoot*m_M + 4*I_swLeg*m_swLeg + 4*I_swLeg*m_swFoot + 4*I_swFoot*m_swLeg + 4*I_swFoot*m_swFoot + 4*m_M*m_swFoot*r^2 + 4*m_swLeg*m_swFoot*r^2 + L_thigh^2*m_M*m_swLeg + 4*L_thigh^2*m_M*m_swFoot + L_thigh^2*m_swLeg*m_swFoot + 8*L_thigh*m_M*m_swFoot*r + 4*L_thigh*m_swLeg*m_swFoot*r)) + (del_y_M_star*(2*L0_ss*L_thigh^2*k0_ss*m_swLeg^2*x_M - 2*L_thigh^2*k0_ss*m_swLeg^2*x_M*(x_M^2 + y_M^2)^(1/2) + 8*I_swLeg*L0_ss*k0_ss*m_M*x_M + 8*I_swFoot*L0_ss*k0_ss*m_M*x_M + 8*I_swLeg*L0_ss*k0_ss*m_swLeg*x_M + 8*I_swFoot*L0_ss*k0_ss*m_swLeg*x_M - 8*I_swLeg*k0_ss*m_M*x_M*(x_M^2 + y_M^2)^(1/2) - 8*I_swFoot*k0_ss*m_M*x_M*(x_M^2 + y_M^2)^(1/2) - 8*I_swLeg*k0_ss*m_swLeg*x_M*(x_M^2 + y_M^2)^(1/2) - 8*I_swFoot*k0_ss*m_swLeg*x_M*(x_M^2 + y_M^2)^(1/2) + 2*L0_ss*L_thigh^2*k0_ss*m_M*m_swLeg*x_M + 8*L0_ss*L_thigh^2*k0_ss*m_M*m_swFoot*x_M + 8*L0_ss*L_thigh^2*k0_ss*m_swLeg*m_swFoot*x_M - 2*L_thigh^2*k0_ss*m_M*m_swLeg*x_M*(x_M^2 + y_M^2)^(1/2) - 8*L_thigh^2*k0_ss*m_M*m_swFoot*x_M*(x_M^2 + y_M^2)^(1/2) - 8*L_thigh^2*k0_ss*m_swLeg*m_swFoot*x_M*(x_M^2 + y_M^2)^(1/2) + 8*I_swLeg*k_swFoot*m_M*r*cos(theta)*(x_M^2 + y_M^2)^(1/2) - 8*I_swLeg*k_swFoot*m_M*r0*cos(theta)*(x_M^2 + y_M^2)^(1/2) + 8*I_swFoot*k_swFoot*m_M*r*cos(theta)*(x_M^2 + y_M^2)^(1/2) - 8*I_swFoot*k_swFoot*m_M*r0*cos(theta)*(x_M^2 + y_M^2)^(1/2) + 8*I_swLeg*k_swFoot*m_swLeg*r*cos(theta)*(x_M^2 + y_M^2)^(1/2) - 8*I_swLeg*k_swFoot*m_swLeg*r0*cos(theta)*(x_M^2 + y_M^2)^(1/2) + 8*I_swLeg*k_swFoot*m_swFoot*r*cos(theta)*(x_M^2 + y_M^2)^(1/2) - 8*I_swLeg*k_swFoot*m_swFoot*r0*cos(theta)*(x_M^2 + y_M^2)^(1/2) + 8*I_swFoot*k_swFoot*m_swLeg*r*cos(theta)*(x_M^2 + y_M^2)^(1/2) - 8*I_swFoot*k_swFoot*m_swLeg*r0*cos(theta)*(x_M^2 + y_M^2)^(1/2) + 8*I_swFoot*k_swFoot*m_swFoot*r*cos(theta)*(x_M^2 + y_M^2)^(1/2) - 8*I_swFoot*k_swFoot*m_swFoot*r0*cos(theta)*(x_M^2 + y_M^2)^(1/2) + 8*L0_ss*k0_ss*m_M*m_swFoot*r^2*x_M + 8*L0_ss*k0_ss*m_swLeg*m_swFoot*r^2*x_M - 2*L0_ss*L_thigh^2*k0_ss*m_swLeg^2*x_M*cos(theta)^2 - L0_ss*L_thigh^2*k0_ss*m_swLeg^2*y_M*sin(2*theta) + L_thigh^3*dtheta^2*m_M*m_swLeg^2*cos(theta)*(x_M^2 + y_M^2)^(1/2) + L_thigh^3*dtheta^2*m_swLeg^2*m_swFoot*cos(theta)*(x_M^2 + y_M^2)^(1/2) - 8*k0_ss*m_M*m_swFoot*r^2*x_M*(x_M^2 + y_M^2)^(1/2) - 8*k0_ss*m_swLeg*m_swFoot*r^2*x_M*(x_M^2 + y_M^2)^(1/2) + 2*L_thigh^2*k0_ss*m_swLeg^2*x_M*cos(theta)^2*(x_M^2 + y_M^2)^(1/2) + L_thigh^2*k0_ss*m_swLeg^2*y_M*sin(2*theta)*(x_M^2 + y_M^2)^(1/2) + 8*I_swLeg*L0_ss*k0_ss*m_swFoot*x_M*cos(theta)^2 + 8*I_swFoot*L0_ss*k0_ss*m_swFoot*x_M*cos(theta)^2 + 4*I_swLeg*L0_ss*k0_ss*m_swFoot*y_M*sin(2*theta) + 4*I_swFoot*L0_ss*k0_ss*m_swFoot*y_M*sin(2*theta) - 8*I_swLeg*k0_ss*m_swFoot*x_M*cos(theta)^2*(x_M^2 + y_M^2)^(1/2) - 8*I_swFoot*k0_ss*m_swFoot*x_M*cos(theta)^2*(x_M^2 + y_M^2)^(1/2) - 4*L_thigh*k_swLeg*m_swLeg^2*theta*sin(theta)*(x_M^2 + y_M^2)^(1/2) + 4*L_thigh*k_swLeg*m_swLeg^2*theta0*sin(theta)*(x_M^2 + y_M^2)^(1/2) - 4*I_swLeg*k0_ss*m_swFoot*y_M*sin(2*theta)*(x_M^2 + y_M^2)^(1/2) - 4*I_swFoot*k0_ss*m_swFoot*y_M*sin(2*theta)*(x_M^2 + y_M^2)^(1/2) + 8*k_swFoot*m_M*m_swFoot*r^3*cos(theta)*(x_M^2 + y_M^2)^(1/2) + 8*k_swFoot*m_swLeg*m_swFoot*r^3*cos(theta)*(x_M^2 + y_M^2)^(1/2) + 4*I_swLeg*L_thigh*dtheta^2*m_swLeg^2*cos(theta)*(x_M^2 + y_M^2)^(1/2) + 4*I_swFoot*L_thigh*dtheta^2*m_swLeg^2*cos(theta)*(x_M^2 + y_M^2)^(1/2) + 2*L_thigh^2*k_swFoot*m_M*m_swLeg*r*cos(theta)*(x_M^2 + y_M^2)^(1/2) - 2*L_thigh^2*k_swFoot*m_M*m_swLeg*r0*cos(theta)*(x_M^2 + y_M^2)^(1/2) + 16*L_thigh*k_swFoot*m_M*m_swFoot*r^2*cos(theta)*(x_M^2 + y_M^2)^(1/2) + 8*L_thigh^2*k_swFoot*m_M*m_swFoot*r*cos(theta)*(x_M^2 + y_M^2)^(1/2) - 8*L_thigh^2*k_swFoot*m_M*m_swFoot*r0*cos(theta)*(x_M^2 + y_M^2)^(1/2) + 8*L_thigh*k_swFoot*m_swLeg*m_swFoot*r^2*cos(theta)*(x_M^2 + y_M^2)^(1/2) + 2*L_thigh^2*k_swFoot*m_swLeg*m_swFoot*r*cos(theta)*(x_M^2 + y_M^2)^(1/2) - 2*L_thigh^2*k_swFoot*m_swLeg*m_swFoot*r0*cos(theta)*(x_M^2 + y_M^2)^(1/2) + 16*L0_ss*L_thigh*k0_ss*m_M*m_swFoot*r*x_M + 16*L0_ss*L_thigh*k0_ss*m_swLeg*m_swFoot*r*x_M - 8*k_swFoot*m_M*m_swFoot*r^2*r0*cos(theta)*(x_M^2 + y_M^2)^(1/2) - 8*k_swFoot*m_swLeg*m_swFoot*r^2*r0*cos(theta)*(x_M^2 + y_M^2)^(1/2) - 16*L_thigh*k0_ss*m_M*m_swFoot*r*x_M*(x_M^2 + y_M^2)^(1/2) - 16*L_thigh*k0_ss*m_swLeg*m_swFoot*r*x_M*(x_M^2 + y_M^2)^(1/2) - 6*L0_ss*L_thigh^2*k0_ss*m_swLeg*m_swFoot*x_M*cos(theta)^2 - 3*L0_ss*L_thigh^2*k0_ss*m_swLeg*m_swFoot*y_M*sin(2*theta) + 4*L_thigh^3*dtheta^2*m_M*m_swLeg*m_swFoot*cos(theta)*(x_M^2 + y_M^2)^(1/2) - 4*L_thigh^2*dr*dtheta*m_swLeg^2*m_swFoot*sin(theta)*(x_M^2 + y_M^2)^(1/2) + 6*L_thigh^2*k0_ss*m_swLeg*m_swFoot*x_M*cos(theta)^2*(x_M^2 + y_M^2)^(1/2) + 3*L_thigh^2*k0_ss*m_swLeg*m_swFoot*y_M*sin(2*theta)*(x_M^2 + y_M^2)^(1/2) + 16*I_swLeg*dr*dtheta*m_M*m_swFoot*sin(theta)*(x_M^2 + y_M^2)^(1/2) + 16*I_swFoot*dr*dtheta*m_M*m_swFoot*sin(theta)*(x_M^2 + y_M^2)^(1/2) + 16*I_swLeg*dr*dtheta*m_swLeg*m_swFoot*sin(theta)*(x_M^2 + y_M^2)^(1/2) + 16*I_swFoot*dr*dtheta*m_swLeg*m_swFoot*sin(theta)*(x_M^2 + y_M^2)^(1/2) - 4*L_thigh*k_swLeg*m_M*m_swLeg*theta*sin(theta)*(x_M^2 + y_M^2)^(1/2) + 4*L_thigh*k_swLeg*m_M*m_swLeg*theta0*sin(theta)*(x_M^2 + y_M^2)^(1/2) - 8*L_thigh*k_swLeg*m_M*m_swFoot*theta*sin(theta)*(x_M^2 + y_M^2)^(1/2) + 8*L_thigh*k_swLeg*m_M*m_swFoot*theta0*sin(theta)*(x_M^2 + y_M^2)^(1/2) - 8*L_thigh*k_swLeg*m_swLeg*m_swFoot*theta*sin(theta)*(x_M^2 + y_M^2)^(1/2) + 8*L_thigh*k_swLeg*m_swLeg*m_swFoot*theta0*sin(theta)*(x_M^2 + y_M^2)^(1/2) + 4*L_thigh*dtheta^2*m_swLeg^2*m_swFoot*r^2*cos(theta)*(x_M^2 + y_M^2)^(1/2) + 4*L_thigh^2*dtheta^2*m_swLeg^2*m_swFoot*r*cos(theta)*(x_M^2 + y_M^2)^(1/2) + 4*I_swLeg*L_thigh*dtheta^2*m_M*m_swLeg*cos(theta)*(x_M^2 + y_M^2)^(1/2) + 4*I_swFoot*L_thigh*dtheta^2*m_M*m_swLeg*cos(theta)*(x_M^2 + y_M^2)^(1/2) + 4*I_swLeg*L_thigh*dtheta^2*m_swLeg*m_swFoot*cos(theta)*(x_M^2 + y_M^2)^(1/2) + 4*I_swFoot*L_thigh*dtheta^2*m_swLeg*m_swFoot*cos(theta)*(x_M^2 + y_M^2)^(1/2) - 8*k_swLeg*m_M*m_swFoot*r*theta*sin(theta)*(x_M^2 + y_M^2)^(1/2) + 8*k_swLeg*m_M*m_swFoot*r*theta0*sin(theta)*(x_M^2 + y_M^2)^(1/2) - 8*k_swLeg*m_swLeg*m_swFoot*r*theta*sin(theta)*(x_M^2 + y_M^2)^(1/2) + 8*k_swLeg*m_swLeg*m_swFoot*r*theta0*sin(theta)*(x_M^2 + y_M^2)^(1/2) - 16*L_thigh*k_swFoot*m_M*m_swFoot*r*r0*cos(theta)*(x_M^2 + y_M^2)^(1/2) - 8*L_thigh*k_swFoot*m_swLeg*m_swFoot*r*r0*cos(theta)*(x_M^2 + y_M^2)^(1/2) - 8*L0_ss*L_thigh*k0_ss*m_swLeg*m_swFoot*r*x_M*cos(theta)^2 - 4*L0_ss*L_thigh*k0_ss*m_swLeg*m_swFoot*r*y_M*sin(2*theta) - 4*L_thigh^2*dr*dtheta*m_M*m_swLeg*m_swFoot*sin(theta)*(x_M^2 + y_M^2)^(1/2) - 8*L_thigh*dr*dtheta*m_swLeg^2*m_swFoot*r*sin(theta)*(x_M^2 + y_M^2)^(1/2) + 8*L_thigh*k0_ss*m_swLeg*m_swFoot*r*x_M*cos(theta)^2*(x_M^2 + y_M^2)^(1/2) + 4*L_thigh*k0_ss*m_swLeg*m_swFoot*r*y_M*sin(2*theta)*(x_M^2 + y_M^2)^(1/2) + 4*L_thigh*dtheta^2*m_M*m_swLeg*m_swFoot*r^2*cos(theta)*(x_M^2 + y_M^2)^(1/2) + 8*L_thigh^2*dtheta^2*m_M*m_swLeg*m_swFoot*r*cos(theta)*(x_M^2 + y_M^2)^(1/2) - 8*L_thigh*dr*dtheta*m_M*m_swLeg*m_swFoot*r*sin(theta)*(x_M^2 + y_M^2)^(1/2)))/(2*(x_M^2 + y_M^2)^(1/2)*(m_M + m_swLeg)*(4*I_swLeg*m_M + 4*I_swFoot*m_M + 4*I_swLeg*m_swLeg + 4*I_swLeg*m_swFoot + 4*I_swFoot*m_swLeg + 4*I_swFoot*m_swFoot + 4*m_M*m_swFoot*r^2 + 4*m_swLeg*m_swFoot*r^2 + L_thigh^2*m_M*m_swLeg + 4*L_thigh^2*m_M*m_swFoot + L_thigh^2*m_swLeg*m_swFoot + 8*L_thigh*m_M*m_swFoot*r + 4*L_thigh*m_swLeg*m_swFoot*r));
                del2_x_swFoot_star*dx_M^2 + dtheta*(dr*sin(theta) + dtheta*cos(theta)*(L_thigh + r)) - K_p*(x_M - x_swFoot_star + cos(theta)*(L_thigh + r)) + K_d*(dx_M*(del_x_swFoot_star - 1) - dr*cos(theta) + dtheta*sin(theta)*(L_thigh + r)) + dr*dtheta*sin(theta) + ((del_x_swFoot_star - 1)*(2*L0_ss*L_thigh^2*k0_ss*m_swLeg^2*x_M - 2*L_thigh^2*k0_ss*m_swLeg^2*x_M*(x_M^2 + y_M^2)^(1/2) + 8*I_swLeg*L0_ss*k0_ss*m_M*x_M + 8*I_swFoot*L0_ss*k0_ss*m_M*x_M + 8*I_swLeg*L0_ss*k0_ss*m_swLeg*x_M + 8*I_swFoot*L0_ss*k0_ss*m_swLeg*x_M - 8*I_swLeg*k0_ss*m_M*x_M*(x_M^2 + y_M^2)^(1/2) - 8*I_swFoot*k0_ss*m_M*x_M*(x_M^2 + y_M^2)^(1/2) - 8*I_swLeg*k0_ss*m_swLeg*x_M*(x_M^2 + y_M^2)^(1/2) - 8*I_swFoot*k0_ss*m_swLeg*x_M*(x_M^2 + y_M^2)^(1/2) + 2*L0_ss*L_thigh^2*k0_ss*m_M*m_swLeg*x_M + 8*L0_ss*L_thigh^2*k0_ss*m_M*m_swFoot*x_M + 8*L0_ss*L_thigh^2*k0_ss*m_swLeg*m_swFoot*x_M - 2*L_thigh^2*k0_ss*m_M*m_swLeg*x_M*(x_M^2 + y_M^2)^(1/2) - 8*L_thigh^2*k0_ss*m_M*m_swFoot*x_M*(x_M^2 + y_M^2)^(1/2) - 8*L_thigh^2*k0_ss*m_swLeg*m_swFoot*x_M*(x_M^2 + y_M^2)^(1/2) + 8*I_swLeg*k_swFoot*m_M*r*cos(theta)*(x_M^2 + y_M^2)^(1/2) - 8*I_swLeg*k_swFoot*m_M*r0*cos(theta)*(x_M^2 + y_M^2)^(1/2) + 8*I_swFoot*k_swFoot*m_M*r*cos(theta)*(x_M^2 + y_M^2)^(1/2) - 8*I_swFoot*k_swFoot*m_M*r0*cos(theta)*(x_M^2 + y_M^2)^(1/2) + 8*I_swLeg*k_swFoot*m_swLeg*r*cos(theta)*(x_M^2 + y_M^2)^(1/2) - 8*I_swLeg*k_swFoot*m_swLeg*r0*cos(theta)*(x_M^2 + y_M^2)^(1/2) + 8*I_swLeg*k_swFoot*m_swFoot*r*cos(theta)*(x_M^2 + y_M^2)^(1/2) - 8*I_swLeg*k_swFoot*m_swFoot*r0*cos(theta)*(x_M^2 + y_M^2)^(1/2) + 8*I_swFoot*k_swFoot*m_swLeg*r*cos(theta)*(x_M^2 + y_M^2)^(1/2) - 8*I_swFoot*k_swFoot*m_swLeg*r0*cos(theta)*(x_M^2 + y_M^2)^(1/2) + 8*I_swFoot*k_swFoot*m_swFoot*r*cos(theta)*(x_M^2 + y_M^2)^(1/2) - 8*I_swFoot*k_swFoot*m_swFoot*r0*cos(theta)*(x_M^2 + y_M^2)^(1/2) + 8*L0_ss*k0_ss*m_M*m_swFoot*r^2*x_M + 8*L0_ss*k0_ss*m_swLeg*m_swFoot*r^2*x_M - 2*L0_ss*L_thigh^2*k0_ss*m_swLeg^2*x_M*cos(theta)^2 - L0_ss*L_thigh^2*k0_ss*m_swLeg^2*y_M*sin(2*theta) + L_thigh^3*dtheta^2*m_M*m_swLeg^2*cos(theta)*(x_M^2 + y_M^2)^(1/2) + L_thigh^3*dtheta^2*m_swLeg^2*m_swFoot*cos(theta)*(x_M^2 + y_M^2)^(1/2) - 8*k0_ss*m_M*m_swFoot*r^2*x_M*(x_M^2 + y_M^2)^(1/2) - 8*k0_ss*m_swLeg*m_swFoot*r^2*x_M*(x_M^2 + y_M^2)^(1/2) + 2*L_thigh^2*k0_ss*m_swLeg^2*x_M*cos(theta)^2*(x_M^2 + y_M^2)^(1/2) + L_thigh^2*k0_ss*m_swLeg^2*y_M*sin(2*theta)*(x_M^2 + y_M^2)^(1/2) + 8*I_swLeg*L0_ss*k0_ss*m_swFoot*x_M*cos(theta)^2 + 8*I_swFoot*L0_ss*k0_ss*m_swFoot*x_M*cos(theta)^2 + 4*I_swLeg*L0_ss*k0_ss*m_swFoot*y_M*sin(2*theta) + 4*I_swFoot*L0_ss*k0_ss*m_swFoot*y_M*sin(2*theta) - 8*I_swLeg*k0_ss*m_swFoot*x_M*cos(theta)^2*(x_M^2 + y_M^2)^(1/2) - 8*I_swFoot*k0_ss*m_swFoot*x_M*cos(theta)^2*(x_M^2 + y_M^2)^(1/2) - 4*L_thigh*k_swLeg*m_swLeg^2*theta*sin(theta)*(x_M^2 + y_M^2)^(1/2) + 4*L_thigh*k_swLeg*m_swLeg^2*theta0*sin(theta)*(x_M^2 + y_M^2)^(1/2) - 4*I_swLeg*k0_ss*m_swFoot*y_M*sin(2*theta)*(x_M^2 + y_M^2)^(1/2) - 4*I_swFoot*k0_ss*m_swFoot*y_M*sin(2*theta)*(x_M^2 + y_M^2)^(1/2) + 8*k_swFoot*m_M*m_swFoot*r^3*cos(theta)*(x_M^2 + y_M^2)^(1/2) + 8*k_swFoot*m_swLeg*m_swFoot*r^3*cos(theta)*(x_M^2 + y_M^2)^(1/2) + 4*I_swLeg*L_thigh*dtheta^2*m_swLeg^2*cos(theta)*(x_M^2 + y_M^2)^(1/2) + 4*I_swFoot*L_thigh*dtheta^2*m_swLeg^2*cos(theta)*(x_M^2 + y_M^2)^(1/2) + 2*L_thigh^2*k_swFoot*m_M*m_swLeg*r*cos(theta)*(x_M^2 + y_M^2)^(1/2) - 2*L_thigh^2*k_swFoot*m_M*m_swLeg*r0*cos(theta)*(x_M^2 + y_M^2)^(1/2) + 16*L_thigh*k_swFoot*m_M*m_swFoot*r^2*cos(theta)*(x_M^2 + y_M^2)^(1/2) + 8*L_thigh^2*k_swFoot*m_M*m_swFoot*r*cos(theta)*(x_M^2 + y_M^2)^(1/2) - 8*L_thigh^2*k_swFoot*m_M*m_swFoot*r0*cos(theta)*(x_M^2 + y_M^2)^(1/2) + 8*L_thigh*k_swFoot*m_swLeg*m_swFoot*r^2*cos(theta)*(x_M^2 + y_M^2)^(1/2) + 2*L_thigh^2*k_swFoot*m_swLeg*m_swFoot*r*cos(theta)*(x_M^2 + y_M^2)^(1/2) - 2*L_thigh^2*k_swFoot*m_swLeg*m_swFoot*r0*cos(theta)*(x_M^2 + y_M^2)^(1/2) + 16*L0_ss*L_thigh*k0_ss*m_M*m_swFoot*r*x_M + 16*L0_ss*L_thigh*k0_ss*m_swLeg*m_swFoot*r*x_M - 8*k_swFoot*m_M*m_swFoot*r^2*r0*cos(theta)*(x_M^2 + y_M^2)^(1/2) - 8*k_swFoot*m_swLeg*m_swFoot*r^2*r0*cos(theta)*(x_M^2 + y_M^2)^(1/2) - 16*L_thigh*k0_ss*m_M*m_swFoot*r*x_M*(x_M^2 + y_M^2)^(1/2) - 16*L_thigh*k0_ss*m_swLeg*m_swFoot*r*x_M*(x_M^2 + y_M^2)^(1/2) - 6*L0_ss*L_thigh^2*k0_ss*m_swLeg*m_swFoot*x_M*cos(theta)^2 - 3*L0_ss*L_thigh^2*k0_ss*m_swLeg*m_swFoot*y_M*sin(2*theta) + 4*L_thigh^3*dtheta^2*m_M*m_swLeg*m_swFoot*cos(theta)*(x_M^2 + y_M^2)^(1/2) - 4*L_thigh^2*dr*dtheta*m_swLeg^2*m_swFoot*sin(theta)*(x_M^2 + y_M^2)^(1/2) + 6*L_thigh^2*k0_ss*m_swLeg*m_swFoot*x_M*cos(theta)^2*(x_M^2 + y_M^2)^(1/2) + 3*L_thigh^2*k0_ss*m_swLeg*m_swFoot*y_M*sin(2*theta)*(x_M^2 + y_M^2)^(1/2) + 16*I_swLeg*dr*dtheta*m_M*m_swFoot*sin(theta)*(x_M^2 + y_M^2)^(1/2) + 16*I_swFoot*dr*dtheta*m_M*m_swFoot*sin(theta)*(x_M^2 + y_M^2)^(1/2) + 16*I_swLeg*dr*dtheta*m_swLeg*m_swFoot*sin(theta)*(x_M^2 + y_M^2)^(1/2) + 16*I_swFoot*dr*dtheta*m_swLeg*m_swFoot*sin(theta)*(x_M^2 + y_M^2)^(1/2) - 4*L_thigh*k_swLeg*m_M*m_swLeg*theta*sin(theta)*(x_M^2 + y_M^2)^(1/2) + 4*L_thigh*k_swLeg*m_M*m_swLeg*theta0*sin(theta)*(x_M^2 + y_M^2)^(1/2) - 8*L_thigh*k_swLeg*m_M*m_swFoot*theta*sin(theta)*(x_M^2 + y_M^2)^(1/2) + 8*L_thigh*k_swLeg*m_M*m_swFoot*theta0*sin(theta)*(x_M^2 + y_M^2)^(1/2) - 8*L_thigh*k_swLeg*m_swLeg*m_swFoot*theta*sin(theta)*(x_M^2 + y_M^2)^(1/2) + 8*L_thigh*k_swLeg*m_swLeg*m_swFoot*theta0*sin(theta)*(x_M^2 + y_M^2)^(1/2) + 4*L_thigh*dtheta^2*m_swLeg^2*m_swFoot*r^2*cos(theta)*(x_M^2 + y_M^2)^(1/2) + 4*L_thigh^2*dtheta^2*m_swLeg^2*m_swFoot*r*cos(theta)*(x_M^2 + y_M^2)^(1/2) + 4*I_swLeg*L_thigh*dtheta^2*m_M*m_swLeg*cos(theta)*(x_M^2 + y_M^2)^(1/2) + 4*I_swFoot*L_thigh*dtheta^2*m_M*m_swLeg*cos(theta)*(x_M^2 + y_M^2)^(1/2) + 4*I_swLeg*L_thigh*dtheta^2*m_swLeg*m_swFoot*cos(theta)*(x_M^2 + y_M^2)^(1/2) + 4*I_swFoot*L_thigh*dtheta^2*m_swLeg*m_swFoot*cos(theta)*(x_M^2 + y_M^2)^(1/2) - 8*k_swLeg*m_M*m_swFoot*r*theta*sin(theta)*(x_M^2 + y_M^2)^(1/2) + 8*k_swLeg*m_M*m_swFoot*r*theta0*sin(theta)*(x_M^2 + y_M^2)^(1/2) - 8*k_swLeg*m_swLeg*m_swFoot*r*theta*sin(theta)*(x_M^2 + y_M^2)^(1/2) + 8*k_swLeg*m_swLeg*m_swFoot*r*theta0*sin(theta)*(x_M^2 + y_M^2)^(1/2) - 16*L_thigh*k_swFoot*m_M*m_swFoot*r*r0*cos(theta)*(x_M^2 + y_M^2)^(1/2) - 8*L_thigh*k_swFoot*m_swLeg*m_swFoot*r*r0*cos(theta)*(x_M^2 + y_M^2)^(1/2) - 8*L0_ss*L_thigh*k0_ss*m_swLeg*m_swFoot*r*x_M*cos(theta)^2 - 4*L0_ss*L_thigh*k0_ss*m_swLeg*m_swFoot*r*y_M*sin(2*theta) - 4*L_thigh^2*dr*dtheta*m_M*m_swLeg*m_swFoot*sin(theta)*(x_M^2 + y_M^2)^(1/2) - 8*L_thigh*dr*dtheta*m_swLeg^2*m_swFoot*r*sin(theta)*(x_M^2 + y_M^2)^(1/2) + 8*L_thigh*k0_ss*m_swLeg*m_swFoot*r*x_M*cos(theta)^2*(x_M^2 + y_M^2)^(1/2) + 4*L_thigh*k0_ss*m_swLeg*m_swFoot*r*y_M*sin(2*theta)*(x_M^2 + y_M^2)^(1/2) + 4*L_thigh*dtheta^2*m_M*m_swLeg*m_swFoot*r^2*cos(theta)*(x_M^2 + y_M^2)^(1/2) + 8*L_thigh^2*dtheta^2*m_M*m_swLeg*m_swFoot*r*cos(theta)*(x_M^2 + y_M^2)^(1/2) - 8*L_thigh*dr*dtheta*m_M*m_swLeg*m_swFoot*r*sin(theta)*(x_M^2 + y_M^2)^(1/2)))/(2*(x_M^2 + y_M^2)^(1/2)*(m_M + m_swLeg)*(4*I_swLeg*m_M + 4*I_swFoot*m_M + 4*I_swLeg*m_swLeg + 4*I_swLeg*m_swFoot + 4*I_swFoot*m_swLeg + 4*I_swFoot*m_swFoot + 4*m_M*m_swFoot*r^2 + 4*m_swLeg*m_swFoot*r^2 + L_thigh^2*m_M*m_swLeg + 4*L_thigh^2*m_M*m_swFoot + L_thigh^2*m_swLeg*m_swFoot + 8*L_thigh*m_M*m_swFoot*r + 4*L_thigh*m_swLeg*m_swFoot*r)) - (sin(theta)*(L_thigh + r)*(4*k_swLeg*m_M*theta*(x_M^2 + y_M^2)^(1/2) - 4*k_swLeg*m_M*theta0*(x_M^2 + y_M^2)^(1/2) + 4*k_swLeg*m_swLeg*theta*(x_M^2 + y_M^2)^(1/2) - 4*k_swLeg*m_swLeg*theta0*(x_M^2 + y_M^2)^(1/2) + 4*k_swLeg*m_swFoot*theta*(x_M^2 + y_M^2)^(1/2) - 4*k_swLeg*m_swFoot*theta0*(x_M^2 + y_M^2)^(1/2) + 2*L0_ss*L_thigh*k0_ss*m_swLeg*y_M*cos(theta) + 4*L0_ss*L_thigh*k0_ss*m_swFoot*y_M*cos(theta) - 2*L0_ss*L_thigh*k0_ss*m_swLeg*x_M*sin(theta) - 4*L0_ss*L_thigh*k0_ss*m_swFoot*x_M*sin(theta) - 2*L_thigh*k0_ss*m_swLeg*y_M*cos(theta)*(x_M^2 + y_M^2)^(1/2) - 4*L_thigh*k0_ss*m_swFoot*y_M*cos(theta)*(x_M^2 + y_M^2)^(1/2) + 4*L0_ss*k0_ss*m_swFoot*r*y_M*cos(theta) + 2*L_thigh*k0_ss*m_swLeg*x_M*sin(theta)*(x_M^2 + y_M^2)^(1/2) + 4*L_thigh*k0_ss*m_swFoot*x_M*sin(theta)*(x_M^2 + y_M^2)^(1/2) - 4*L0_ss*k0_ss*m_swFoot*r*x_M*sin(theta) - 4*k0_ss*m_swFoot*r*y_M*cos(theta)*(x_M^2 + y_M^2)^(1/2) + 4*k0_ss*m_swFoot*r*x_M*sin(theta)*(x_M^2 + y_M^2)^(1/2) + 8*L_thigh*dr*dtheta*m_M*m_swFoot*(x_M^2 + y_M^2)^(1/2) + 4*L_thigh*dr*dtheta*m_swLeg*m_swFoot*(x_M^2 + y_M^2)^(1/2) + 8*dr*dtheta*m_M*m_swFoot*r*(x_M^2 + y_M^2)^(1/2) + 8*dr*dtheta*m_swLeg*m_swFoot*r*(x_M^2 + y_M^2)^(1/2)))/((x_M^2 + y_M^2)^(1/2)*(4*I_swLeg*m_M + 4*I_swFoot*m_M + 4*I_swLeg*m_swLeg + 4*I_swLeg*m_swFoot + 4*I_swFoot*m_swLeg + 4*I_swFoot*m_swFoot + 4*m_M*m_swFoot*r^2 + 4*m_swLeg*m_swFoot*r^2 + L_thigh^2*m_M*m_swLeg + 4*L_thigh^2*m_M*m_swFoot + L_thigh^2*m_swLeg*m_swFoot + 8*L_thigh*m_M*m_swFoot*r + 4*L_thigh*m_swLeg*m_swFoot*r)) - (cos(theta)*(2*k_swFoot*m_M*r0*(x_M^2 + y_M^2)^(1/2) - 2*k_swFoot*m_M*r*(x_M^2 + y_M^2)^(1/2) - 2*k_swFoot*m_swLeg*r*(x_M^2 + y_M^2)^(1/2) + 2*k_swFoot*m_swLeg*r0*(x_M^2 + y_M^2)^(1/2) - 2*k_swFoot*m_swFoot*r*(x_M^2 + y_M^2)^(1/2) + 2*k_swFoot*m_swFoot*r0*(x_M^2 + y_M^2)^(1/2) + 2*k0_ss*m_swFoot*y_M*sin(theta)*(x_M^2 + y_M^2)^(1/2) + 2*L_thigh*dtheta^2*m_M*m_swFoot*(x_M^2 + y_M^2)^(1/2) + L_thigh*dtheta^2*m_swLeg*m_swFoot*(x_M^2 + y_M^2)^(1/2) - 2*L0_ss*k0_ss*m_swFoot*x_M*cos(theta) + 2*dtheta^2*m_M*m_swFoot*r*(x_M^2 + y_M^2)^(1/2) + 2*dtheta^2*m_swLeg*m_swFoot*r*(x_M^2 + y_M^2)^(1/2) - 2*L0_ss*k0_ss*m_swFoot*y_M*sin(theta) + 2*k0_ss*m_swFoot*x_M*cos(theta)*(x_M^2 + y_M^2)^(1/2)))/(2*m_swFoot*(x_M^2 + y_M^2)^(1/2)*(m_M + m_swLeg));
                del2_y_swFoot_star*dx_M^2 - dtheta*(dr*cos(theta) - dtheta*sin(theta)*(L_thigh + r)) - K_p*(y_M - y_swFoot_star + sin(theta)*(L_thigh + r)) - K_d*(dy_M - del_y_swFoot_star*dx_M + dr*sin(theta) + dtheta*cos(theta)*(L_thigh + r)) - dr*dtheta*cos(theta) + (8*I_swLeg*gravi*m_M^2*(x_M^2 + y_M^2)^(1/2) + 8*I_swFoot*gravi*m_M^2*(x_M^2 + y_M^2)^(1/2) + 8*I_swLeg*gravi*m_swLeg^2*(x_M^2 + y_M^2)^(1/2) + 8*I_swFoot*gravi*m_swLeg^2*(x_M^2 + y_M^2)^(1/2) - L0_ss*L_thigh^2*k0_ss*m_swLeg^2*y_M + 2*L_thigh^2*gravi*m_M*m_swLeg^2*(x_M^2 + y_M^2)^(1/2) + 2*L_thigh^2*gravi*m_M^2*m_swLeg*(x_M^2 + y_M^2)^(1/2) + 8*L_thigh^2*gravi*m_M^2*m_swFoot*(x_M^2 + y_M^2)^(1/2) + 2*L_thigh^2*gravi*m_swLeg^2*m_swFoot*(x_M^2 + y_M^2)^(1/2) + L_thigh^2*k0_ss*m_swLeg^2*y_M*(x_M^2 + y_M^2)^(1/2) + 8*gravi*m_M^2*m_swFoot*r^2*(x_M^2 + y_M^2)^(1/2) + 8*gravi*m_swLeg^2*m_swFoot*r^2*(x_M^2 + y_M^2)^(1/2) - 8*I_swLeg*L0_ss*k0_ss*m_M*y_M - 8*I_swFoot*L0_ss*k0_ss*m_M*y_M - 8*I_swLeg*L0_ss*k0_ss*m_swLeg*y_M - 4*I_swLeg*L0_ss*k0_ss*m_swFoot*y_M - 8*I_swFoot*L0_ss*k0_ss*m_swLeg*y_M - 4*I_swFoot*L0_ss*k0_ss*m_swFoot*y_M + 16*I_swLeg*gravi*m_M*m_swLeg*(x_M^2 + y_M^2)^(1/2) + 8*I_swLeg*gravi*m_M*m_swFoot*(x_M^2 + y_M^2)^(1/2) + 16*I_swFoot*gravi*m_M*m_swLeg*(x_M^2 + y_M^2)^(1/2) + 8*I_swFoot*gravi*m_M*m_swFoot*(x_M^2 + y_M^2)^(1/2) + 8*I_swLeg*gravi*m_swLeg*m_swFoot*(x_M^2 + y_M^2)^(1/2) + 8*I_swFoot*gravi*m_swLeg*m_swFoot*(x_M^2 + y_M^2)^(1/2) + 8*I_swLeg*k0_ss*m_M*y_M*(x_M^2 + y_M^2)^(1/2) + 8*I_swFoot*k0_ss*m_M*y_M*(x_M^2 + y_M^2)^(1/2) + 8*I_swLeg*k0_ss*m_swLeg*y_M*(x_M^2 + y_M^2)^(1/2) + 4*I_swLeg*k0_ss*m_swFoot*y_M*(x_M^2 + y_M^2)^(1/2) + 8*I_swFoot*k0_ss*m_swLeg*y_M*(x_M^2 + y_M^2)^(1/2) + 4*I_swFoot*k0_ss*m_swFoot*y_M*(x_M^2 + y_M^2)^(1/2) - 2*L0_ss*L_thigh^2*k0_ss*m_M*m_swLeg*y_M - 8*L0_ss*L_thigh^2*k0_ss*m_M*m_swFoot*y_M - 5*L0_ss*L_thigh^2*k0_ss*m_swLeg*m_swFoot*y_M + 10*L_thigh^2*gravi*m_M*m_swLeg*m_swFoot*(x_M^2 + y_M^2)^(1/2) + 16*L_thigh*gravi*m_M^2*m_swFoot*r*(x_M^2 + y_M^2)^(1/2) + 8*L_thigh*gravi*m_swLeg^2*m_swFoot*r*(x_M^2 + y_M^2)^(1/2) + 2*L_thigh^2*k0_ss*m_M*m_swLeg*y_M*(x_M^2 + y_M^2)^(1/2) + 8*L_thigh^2*k0_ss*m_M*m_swFoot*y_M*(x_M^2 + y_M^2)^(1/2) + 5*L_thigh^2*k0_ss*m_swLeg*m_swFoot*y_M*(x_M^2 + y_M^2)^(1/2) - 8*L0_ss*k0_ss*m_M*m_swFoot*r^2*y_M - 8*L0_ss*k0_ss*m_swLeg*m_swFoot*r^2*y_M - L0_ss*L_thigh^2*k0_ss*m_swLeg^2*y_M*cos(2*theta) - 8*I_swLeg*k_swFoot*m_M*r*sin(theta)*(x_M^2 + y_M^2)^(1/2) + 8*I_swLeg*k_swFoot*m_M*r0*sin(theta)*(x_M^2 + y_M^2)^(1/2) - 8*I_swFoot*k_swFoot*m_M*r*sin(theta)*(x_M^2 + y_M^2)^(1/2) + 8*I_swFoot*k_swFoot*m_M*r0*sin(theta)*(x_M^2 + y_M^2)^(1/2) - 8*I_swLeg*k_swFoot*m_swLeg*r*sin(theta)*(x_M^2 + y_M^2)^(1/2) + 8*I_swLeg*k_swFoot*m_swLeg*r0*sin(theta)*(x_M^2 + y_M^2)^(1/2) - 8*I_swLeg*k_swFoot*m_swFoot*r*sin(theta)*(x_M^2 + y_M^2)^(1/2) + 8*I_swLeg*k_swFoot*m_swFoot*r0*sin(theta)*(x_M^2 + y_M^2)^(1/2) - 8*I_swFoot*k_swFoot*m_swLeg*r*sin(theta)*(x_M^2 + y_M^2)^(1/2) + 8*I_swFoot*k_swFoot*m_swLeg*r0*sin(theta)*(x_M^2 + y_M^2)^(1/2) - 8*I_swFoot*k_swFoot*m_swFoot*r*sin(theta)*(x_M^2 + y_M^2)^(1/2) + 8*I_swFoot*k_swFoot*m_swFoot*r0*sin(theta)*(x_M^2 + y_M^2)^(1/2) + L0_ss*L_thigh^2*k0_ss*m_swLeg^2*x_M*sin(2*theta) + 16*gravi*m_M*m_swLeg*m_swFoot*r^2*(x_M^2 + y_M^2)^(1/2) + 8*k0_ss*m_M*m_swFoot*r^2*y_M*(x_M^2 + y_M^2)^(1/2) + 8*k0_ss*m_swLeg*m_swFoot*r^2*y_M*(x_M^2 + y_M^2)^(1/2) - L_thigh^3*dtheta^2*m_M*m_swLeg^2*sin(theta)*(x_M^2 + y_M^2)^(1/2) - L_thigh^3*dtheta^2*m_swLeg^2*m_swFoot*sin(theta)*(x_M^2 + y_M^2)^(1/2) + L_thigh^2*k0_ss*m_swLeg^2*y_M*cos(2*theta)*(x_M^2 + y_M^2)^(1/2) - L_thigh^2*k0_ss*m_swLeg^2*x_M*sin(2*theta)*(x_M^2 + y_M^2)^(1/2) + 4*I_swLeg*L0_ss*k0_ss*m_swFoot*y_M*cos(2*theta) + 4*I_swFoot*L0_ss*k0_ss*m_swFoot*y_M*cos(2*theta) - 4*I_swLeg*L0_ss*k0_ss*m_swFoot*x_M*sin(2*theta) - 4*I_swFoot*L0_ss*k0_ss*m_swFoot*x_M*sin(2*theta) - 4*L_thigh*k_swLeg*m_swLeg^2*theta*cos(theta)*(x_M^2 + y_M^2)^(1/2) + 4*L_thigh*k_swLeg*m_swLeg^2*theta0*cos(theta)*(x_M^2 + y_M^2)^(1/2) - 4*I_swLeg*k0_ss*m_swFoot*y_M*cos(2*theta)*(x_M^2 + y_M^2)^(1/2) - 4*I_swFoot*k0_ss*m_swFoot*y_M*cos(2*theta)*(x_M^2 + y_M^2)^(1/2) + 4*I_swLeg*k0_ss*m_swFoot*x_M*sin(2*theta)*(x_M^2 + y_M^2)^(1/2) + 4*I_swFoot*k0_ss*m_swFoot*x_M*sin(2*theta)*(x_M^2 + y_M^2)^(1/2) - 8*k_swFoot*m_M*m_swFoot*r^3*sin(theta)*(x_M^2 + y_M^2)^(1/2) - 8*k_swFoot*m_swLeg*m_swFoot*r^3*sin(theta)*(x_M^2 + y_M^2)^(1/2) - 4*I_swLeg*L_thigh*dtheta^2*m_swLeg^2*sin(theta)*(x_M^2 + y_M^2)^(1/2) - 4*I_swFoot*L_thigh*dtheta^2*m_swLeg^2*sin(theta)*(x_M^2 + y_M^2)^(1/2) - 2*L_thigh^2*k_swFoot*m_M*m_swLeg*r*sin(theta)*(x_M^2 + y_M^2)^(1/2) + 2*L_thigh^2*k_swFoot*m_M*m_swLeg*r0*sin(theta)*(x_M^2 + y_M^2)^(1/2) - 16*L_thigh*k_swFoot*m_M*m_swFoot*r^2*sin(theta)*(x_M^2 + y_M^2)^(1/2) - 8*L_thigh^2*k_swFoot*m_M*m_swFoot*r*sin(theta)*(x_M^2 + y_M^2)^(1/2) + 8*L_thigh^2*k_swFoot*m_M*m_swFoot*r0*sin(theta)*(x_M^2 + y_M^2)^(1/2) - 8*L_thigh*k_swFoot*m_swLeg*m_swFoot*r^2*sin(theta)*(x_M^2 + y_M^2)^(1/2) - 2*L_thigh^2*k_swFoot*m_swLeg*m_swFoot*r*sin(theta)*(x_M^2 + y_M^2)^(1/2) + 2*L_thigh^2*k_swFoot*m_swLeg*m_swFoot*r0*sin(theta)*(x_M^2 + y_M^2)^(1/2) - 16*L0_ss*L_thigh*k0_ss*m_M*m_swFoot*r*y_M - 12*L0_ss*L_thigh*k0_ss*m_swLeg*m_swFoot*r*y_M + 24*L_thigh*gravi*m_M*m_swLeg*m_swFoot*r*(x_M^2 + y_M^2)^(1/2) + 8*k_swFoot*m_M*m_swFoot*r^2*r0*sin(theta)*(x_M^2 + y_M^2)^(1/2) + 8*k_swFoot*m_swLeg*m_swFoot*r^2*r0*sin(theta)*(x_M^2 + y_M^2)^(1/2) + 16*L_thigh*k0_ss*m_M*m_swFoot*r*y_M*(x_M^2 + y_M^2)^(1/2) + 12*L_thigh*k0_ss*m_swLeg*m_swFoot*r*y_M*(x_M^2 + y_M^2)^(1/2) - 3*L0_ss*L_thigh^2*k0_ss*m_swLeg*m_swFoot*y_M*cos(2*theta) - 4*L_thigh^2*dr*dtheta*m_swLeg^2*m_swFoot*cos(theta)*(x_M^2 + y_M^2)^(1/2) + 3*L0_ss*L_thigh^2*k0_ss*m_swLeg*m_swFoot*x_M*sin(2*theta) - 4*L_thigh^3*dtheta^2*m_M*m_swLeg*m_swFoot*sin(theta)*(x_M^2 + y_M^2)^(1/2) + 3*L_thigh^2*k0_ss*m_swLeg*m_swFoot*y_M*cos(2*theta)*(x_M^2 + y_M^2)^(1/2) - 3*L_thigh^2*k0_ss*m_swLeg*m_swFoot*x_M*sin(2*theta)*(x_M^2 + y_M^2)^(1/2) + 16*I_swLeg*dr*dtheta*m_M*m_swFoot*cos(theta)*(x_M^2 + y_M^2)^(1/2) + 16*I_swFoot*dr*dtheta*m_M*m_swFoot*cos(theta)*(x_M^2 + y_M^2)^(1/2) + 16*I_swLeg*dr*dtheta*m_swLeg*m_swFoot*cos(theta)*(x_M^2 + y_M^2)^(1/2) + 16*I_swFoot*dr*dtheta*m_swLeg*m_swFoot*cos(theta)*(x_M^2 + y_M^2)^(1/2) - 4*L_thigh*k_swLeg*m_M*m_swLeg*theta*cos(theta)*(x_M^2 + y_M^2)^(1/2) + 4*L_thigh*k_swLeg*m_M*m_swLeg*theta0*cos(theta)*(x_M^2 + y_M^2)^(1/2) - 8*L_thigh*k_swLeg*m_M*m_swFoot*theta*cos(theta)*(x_M^2 + y_M^2)^(1/2) + 8*L_thigh*k_swLeg*m_M*m_swFoot*theta0*cos(theta)*(x_M^2 + y_M^2)^(1/2) - 8*L_thigh*k_swLeg*m_swLeg*m_swFoot*theta*cos(theta)*(x_M^2 + y_M^2)^(1/2) + 8*L_thigh*k_swLeg*m_swLeg*m_swFoot*theta0*cos(theta)*(x_M^2 + y_M^2)^(1/2) - 4*L_thigh*dtheta^2*m_swLeg^2*m_swFoot*r^2*sin(theta)*(x_M^2 + y_M^2)^(1/2) - 4*L_thigh^2*dtheta^2*m_swLeg^2*m_swFoot*r*sin(theta)*(x_M^2 + y_M^2)^(1/2) - 8*k_swLeg*m_M*m_swFoot*r*theta*cos(theta)*(x_M^2 + y_M^2)^(1/2) + 8*k_swLeg*m_M*m_swFoot*r*theta0*cos(theta)*(x_M^2 + y_M^2)^(1/2) - 8*k_swLeg*m_swLeg*m_swFoot*r*theta*cos(theta)*(x_M^2 + y_M^2)^(1/2) + 8*k_swLeg*m_swLeg*m_swFoot*r*theta0*cos(theta)*(x_M^2 + y_M^2)^(1/2) - 4*I_swLeg*L_thigh*dtheta^2*m_M*m_swLeg*sin(theta)*(x_M^2 + y_M^2)^(1/2) - 4*I_swFoot*L_thigh*dtheta^2*m_M*m_swLeg*sin(theta)*(x_M^2 + y_M^2)^(1/2) - 4*I_swLeg*L_thigh*dtheta^2*m_swLeg*m_swFoot*sin(theta)*(x_M^2 + y_M^2)^(1/2) - 4*I_swFoot*L_thigh*dtheta^2*m_swLeg*m_swFoot*sin(theta)*(x_M^2 + y_M^2)^(1/2) + 16*L_thigh*k_swFoot*m_M*m_swFoot*r*r0*sin(theta)*(x_M^2 + y_M^2)^(1/2) + 8*L_thigh*k_swFoot*m_swLeg*m_swFoot*r*r0*sin(theta)*(x_M^2 + y_M^2)^(1/2) - 4*L0_ss*L_thigh*k0_ss*m_swLeg*m_swFoot*r*y_M*cos(2*theta) - 4*L_thigh^2*dr*dtheta*m_M*m_swLeg*m_swFoot*cos(theta)*(x_M^2 + y_M^2)^(1/2) - 8*L_thigh*dr*dtheta*m_swLeg^2*m_swFoot*r*cos(theta)*(x_M^2 + y_M^2)^(1/2) + 4*L0_ss*L_thigh*k0_ss*m_swLeg*m_swFoot*r*x_M*sin(2*theta) + 4*L_thigh*k0_ss*m_swLeg*m_swFoot*r*y_M*cos(2*theta)*(x_M^2 + y_M^2)^(1/2) - 4*L_thigh*k0_ss*m_swLeg*m_swFoot*r*x_M*sin(2*theta)*(x_M^2 + y_M^2)^(1/2) - 4*L_thigh*dtheta^2*m_M*m_swLeg*m_swFoot*r^2*sin(theta)*(x_M^2 + y_M^2)^(1/2) - 8*L_thigh^2*dtheta^2*m_M*m_swLeg*m_swFoot*r*sin(theta)*(x_M^2 + y_M^2)^(1/2) - 8*L_thigh*dr*dtheta*m_M*m_swLeg*m_swFoot*r*cos(theta)*(x_M^2 + y_M^2)^(1/2))/(2*(x_M^2 + y_M^2)^(1/2)*(m_M + m_swLeg)*(4*I_swLeg*m_M + 4*I_swFoot*m_M + 4*I_swLeg*m_swLeg + 4*I_swLeg*m_swFoot + 4*I_swFoot*m_swLeg + 4*I_swFoot*m_swFoot + 4*m_M*m_swFoot*r^2 + 4*m_swLeg*m_swFoot*r^2 + L_thigh^2*m_M*m_swLeg + 4*L_thigh^2*m_M*m_swFoot + L_thigh^2*m_swLeg*m_swFoot + 8*L_thigh*m_M*m_swFoot*r + 4*L_thigh*m_swLeg*m_swFoot*r)) - (sin(theta)*(2*k_swFoot*m_M*r0*(x_M^2 + y_M^2)^(1/2) - 2*k_swFoot*m_M*r*(x_M^2 + y_M^2)^(1/2) - 2*k_swFoot*m_swLeg*r*(x_M^2 + y_M^2)^(1/2) + 2*k_swFoot*m_swLeg*r0*(x_M^2 + y_M^2)^(1/2) - 2*k_swFoot*m_swFoot*r*(x_M^2 + y_M^2)^(1/2) + 2*k_swFoot*m_swFoot*r0*(x_M^2 + y_M^2)^(1/2) + 2*k0_ss*m_swFoot*y_M*sin(theta)*(x_M^2 + y_M^2)^(1/2) + 2*L_thigh*dtheta^2*m_M*m_swFoot*(x_M^2 + y_M^2)^(1/2) + L_thigh*dtheta^2*m_swLeg*m_swFoot*(x_M^2 + y_M^2)^(1/2) - 2*L0_ss*k0_ss*m_swFoot*x_M*cos(theta) + 2*dtheta^2*m_M*m_swFoot*r*(x_M^2 + y_M^2)^(1/2) + 2*dtheta^2*m_swLeg*m_swFoot*r*(x_M^2 + y_M^2)^(1/2) - 2*L0_ss*k0_ss*m_swFoot*y_M*sin(theta) + 2*k0_ss*m_swFoot*x_M*cos(theta)*(x_M^2 + y_M^2)^(1/2)))/(2*m_swFoot*(x_M^2 + y_M^2)^(1/2)*(m_M + m_swLeg)) + (cos(theta)*(L_thigh + r)*(4*k_swLeg*m_M*theta*(x_M^2 + y_M^2)^(1/2) - 4*k_swLeg*m_M*theta0*(x_M^2 + y_M^2)^(1/2) + 4*k_swLeg*m_swLeg*theta*(x_M^2 + y_M^2)^(1/2) - 4*k_swLeg*m_swLeg*theta0*(x_M^2 + y_M^2)^(1/2) + 4*k_swLeg*m_swFoot*theta*(x_M^2 + y_M^2)^(1/2) - 4*k_swLeg*m_swFoot*theta0*(x_M^2 + y_M^2)^(1/2) + 2*L0_ss*L_thigh*k0_ss*m_swLeg*y_M*cos(theta) + 4*L0_ss*L_thigh*k0_ss*m_swFoot*y_M*cos(theta) - 2*L0_ss*L_thigh*k0_ss*m_swLeg*x_M*sin(theta) - 4*L0_ss*L_thigh*k0_ss*m_swFoot*x_M*sin(theta) - 2*L_thigh*k0_ss*m_swLeg*y_M*cos(theta)*(x_M^2 + y_M^2)^(1/2) - 4*L_thigh*k0_ss*m_swFoot*y_M*cos(theta)*(x_M^2 + y_M^2)^(1/2) + 4*L0_ss*k0_ss*m_swFoot*r*y_M*cos(theta) + 2*L_thigh*k0_ss*m_swLeg*x_M*sin(theta)*(x_M^2 + y_M^2)^(1/2) + 4*L_thigh*k0_ss*m_swFoot*x_M*sin(theta)*(x_M^2 + y_M^2)^(1/2) - 4*L0_ss*k0_ss*m_swFoot*r*x_M*sin(theta) - 4*k0_ss*m_swFoot*r*y_M*cos(theta)*(x_M^2 + y_M^2)^(1/2) + 4*k0_ss*m_swFoot*r*x_M*sin(theta)*(x_M^2 + y_M^2)^(1/2) + 8*L_thigh*dr*dtheta*m_M*m_swFoot*(x_M^2 + y_M^2)^(1/2) + 4*L_thigh*dr*dtheta*m_swLeg*m_swFoot*(x_M^2 + y_M^2)^(1/2) + 8*dr*dtheta*m_M*m_swFoot*r*(x_M^2 + y_M^2)^(1/2) + 8*dr*dtheta*m_swLeg*m_swFoot*r*(x_M^2 + y_M^2)^(1/2)))/((x_M^2 + y_M^2)^(1/2)*(4*I_swLeg*m_M + 4*I_swFoot*m_M + 4*I_swLeg*m_swLeg + 4*I_swLeg*m_swFoot + 4*I_swFoot*m_swLeg + 4*I_swFoot*m_swFoot + 4*m_M*m_swFoot*r^2 + 4*m_swLeg*m_swFoot*r^2 + L_thigh^2*m_M*m_swLeg + 4*L_thigh^2*m_M*m_swFoot + L_thigh^2*m_swLeg*m_swFoot + 8*L_thigh*m_M*m_swFoot*r + 4*L_thigh*m_swLeg*m_swFoot*r)) + (del_y_swFoot_star*(2*L0_ss*L_thigh^2*k0_ss*m_swLeg^2*x_M - 2*L_thigh^2*k0_ss*m_swLeg^2*x_M*(x_M^2 + y_M^2)^(1/2) + 8*I_swLeg*L0_ss*k0_ss*m_M*x_M + 8*I_swFoot*L0_ss*k0_ss*m_M*x_M + 8*I_swLeg*L0_ss*k0_ss*m_swLeg*x_M + 8*I_swFoot*L0_ss*k0_ss*m_swLeg*x_M - 8*I_swLeg*k0_ss*m_M*x_M*(x_M^2 + y_M^2)^(1/2) - 8*I_swFoot*k0_ss*m_M*x_M*(x_M^2 + y_M^2)^(1/2) - 8*I_swLeg*k0_ss*m_swLeg*x_M*(x_M^2 + y_M^2)^(1/2) - 8*I_swFoot*k0_ss*m_swLeg*x_M*(x_M^2 + y_M^2)^(1/2) + 2*L0_ss*L_thigh^2*k0_ss*m_M*m_swLeg*x_M + 8*L0_ss*L_thigh^2*k0_ss*m_M*m_swFoot*x_M + 8*L0_ss*L_thigh^2*k0_ss*m_swLeg*m_swFoot*x_M - 2*L_thigh^2*k0_ss*m_M*m_swLeg*x_M*(x_M^2 + y_M^2)^(1/2) - 8*L_thigh^2*k0_ss*m_M*m_swFoot*x_M*(x_M^2 + y_M^2)^(1/2) - 8*L_thigh^2*k0_ss*m_swLeg*m_swFoot*x_M*(x_M^2 + y_M^2)^(1/2) + 8*I_swLeg*k_swFoot*m_M*r*cos(theta)*(x_M^2 + y_M^2)^(1/2) - 8*I_swLeg*k_swFoot*m_M*r0*cos(theta)*(x_M^2 + y_M^2)^(1/2) + 8*I_swFoot*k_swFoot*m_M*r*cos(theta)*(x_M^2 + y_M^2)^(1/2) - 8*I_swFoot*k_swFoot*m_M*r0*cos(theta)*(x_M^2 + y_M^2)^(1/2) + 8*I_swLeg*k_swFoot*m_swLeg*r*cos(theta)*(x_M^2 + y_M^2)^(1/2) - 8*I_swLeg*k_swFoot*m_swLeg*r0*cos(theta)*(x_M^2 + y_M^2)^(1/2) + 8*I_swLeg*k_swFoot*m_swFoot*r*cos(theta)*(x_M^2 + y_M^2)^(1/2) - 8*I_swLeg*k_swFoot*m_swFoot*r0*cos(theta)*(x_M^2 + y_M^2)^(1/2) + 8*I_swFoot*k_swFoot*m_swLeg*r*cos(theta)*(x_M^2 + y_M^2)^(1/2) - 8*I_swFoot*k_swFoot*m_swLeg*r0*cos(theta)*(x_M^2 + y_M^2)^(1/2) + 8*I_swFoot*k_swFoot*m_swFoot*r*cos(theta)*(x_M^2 + y_M^2)^(1/2) - 8*I_swFoot*k_swFoot*m_swFoot*r0*cos(theta)*(x_M^2 + y_M^2)^(1/2) + 8*L0_ss*k0_ss*m_M*m_swFoot*r^2*x_M + 8*L0_ss*k0_ss*m_swLeg*m_swFoot*r^2*x_M - 2*L0_ss*L_thigh^2*k0_ss*m_swLeg^2*x_M*cos(theta)^2 - L0_ss*L_thigh^2*k0_ss*m_swLeg^2*y_M*sin(2*theta) + L_thigh^3*dtheta^2*m_M*m_swLeg^2*cos(theta)*(x_M^2 + y_M^2)^(1/2) + L_thigh^3*dtheta^2*m_swLeg^2*m_swFoot*cos(theta)*(x_M^2 + y_M^2)^(1/2) - 8*k0_ss*m_M*m_swFoot*r^2*x_M*(x_M^2 + y_M^2)^(1/2) - 8*k0_ss*m_swLeg*m_swFoot*r^2*x_M*(x_M^2 + y_M^2)^(1/2) + 2*L_thigh^2*k0_ss*m_swLeg^2*x_M*cos(theta)^2*(x_M^2 + y_M^2)^(1/2) + L_thigh^2*k0_ss*m_swLeg^2*y_M*sin(2*theta)*(x_M^2 + y_M^2)^(1/2) + 8*I_swLeg*L0_ss*k0_ss*m_swFoot*x_M*cos(theta)^2 + 8*I_swFoot*L0_ss*k0_ss*m_swFoot*x_M*cos(theta)^2 + 4*I_swLeg*L0_ss*k0_ss*m_swFoot*y_M*sin(2*theta) + 4*I_swFoot*L0_ss*k0_ss*m_swFoot*y_M*sin(2*theta) - 8*I_swLeg*k0_ss*m_swFoot*x_M*cos(theta)^2*(x_M^2 + y_M^2)^(1/2) - 8*I_swFoot*k0_ss*m_swFoot*x_M*cos(theta)^2*(x_M^2 + y_M^2)^(1/2) - 4*L_thigh*k_swLeg*m_swLeg^2*theta*sin(theta)*(x_M^2 + y_M^2)^(1/2) + 4*L_thigh*k_swLeg*m_swLeg^2*theta0*sin(theta)*(x_M^2 + y_M^2)^(1/2) - 4*I_swLeg*k0_ss*m_swFoot*y_M*sin(2*theta)*(x_M^2 + y_M^2)^(1/2) - 4*I_swFoot*k0_ss*m_swFoot*y_M*sin(2*theta)*(x_M^2 + y_M^2)^(1/2) + 8*k_swFoot*m_M*m_swFoot*r^3*cos(theta)*(x_M^2 + y_M^2)^(1/2) + 8*k_swFoot*m_swLeg*m_swFoot*r^3*cos(theta)*(x_M^2 + y_M^2)^(1/2) + 4*I_swLeg*L_thigh*dtheta^2*m_swLeg^2*cos(theta)*(x_M^2 + y_M^2)^(1/2) + 4*I_swFoot*L_thigh*dtheta^2*m_swLeg^2*cos(theta)*(x_M^2 + y_M^2)^(1/2) + 2*L_thigh^2*k_swFoot*m_M*m_swLeg*r*cos(theta)*(x_M^2 + y_M^2)^(1/2) - 2*L_thigh^2*k_swFoot*m_M*m_swLeg*r0*cos(theta)*(x_M^2 + y_M^2)^(1/2) + 16*L_thigh*k_swFoot*m_M*m_swFoot*r^2*cos(theta)*(x_M^2 + y_M^2)^(1/2) + 8*L_thigh^2*k_swFoot*m_M*m_swFoot*r*cos(theta)*(x_M^2 + y_M^2)^(1/2) - 8*L_thigh^2*k_swFoot*m_M*m_swFoot*r0*cos(theta)*(x_M^2 + y_M^2)^(1/2) + 8*L_thigh*k_swFoot*m_swLeg*m_swFoot*r^2*cos(theta)*(x_M^2 + y_M^2)^(1/2) + 2*L_thigh^2*k_swFoot*m_swLeg*m_swFoot*r*cos(theta)*(x_M^2 + y_M^2)^(1/2) - 2*L_thigh^2*k_swFoot*m_swLeg*m_swFoot*r0*cos(theta)*(x_M^2 + y_M^2)^(1/2) + 16*L0_ss*L_thigh*k0_ss*m_M*m_swFoot*r*x_M + 16*L0_ss*L_thigh*k0_ss*m_swLeg*m_swFoot*r*x_M - 8*k_swFoot*m_M*m_swFoot*r^2*r0*cos(theta)*(x_M^2 + y_M^2)^(1/2) - 8*k_swFoot*m_swLeg*m_swFoot*r^2*r0*cos(theta)*(x_M^2 + y_M^2)^(1/2) - 16*L_thigh*k0_ss*m_M*m_swFoot*r*x_M*(x_M^2 + y_M^2)^(1/2) - 16*L_thigh*k0_ss*m_swLeg*m_swFoot*r*x_M*(x_M^2 + y_M^2)^(1/2) - 6*L0_ss*L_thigh^2*k0_ss*m_swLeg*m_swFoot*x_M*cos(theta)^2 - 3*L0_ss*L_thigh^2*k0_ss*m_swLeg*m_swFoot*y_M*sin(2*theta) + 4*L_thigh^3*dtheta^2*m_M*m_swLeg*m_swFoot*cos(theta)*(x_M^2 + y_M^2)^(1/2) - 4*L_thigh^2*dr*dtheta*m_swLeg^2*m_swFoot*sin(theta)*(x_M^2 + y_M^2)^(1/2) + 6*L_thigh^2*k0_ss*m_swLeg*m_swFoot*x_M*cos(theta)^2*(x_M^2 + y_M^2)^(1/2) + 3*L_thigh^2*k0_ss*m_swLeg*m_swFoot*y_M*sin(2*theta)*(x_M^2 + y_M^2)^(1/2) + 16*I_swLeg*dr*dtheta*m_M*m_swFoot*sin(theta)*(x_M^2 + y_M^2)^(1/2) + 16*I_swFoot*dr*dtheta*m_M*m_swFoot*sin(theta)*(x_M^2 + y_M^2)^(1/2) + 16*I_swLeg*dr*dtheta*m_swLeg*m_swFoot*sin(theta)*(x_M^2 + y_M^2)^(1/2) + 16*I_swFoot*dr*dtheta*m_swLeg*m_swFoot*sin(theta)*(x_M^2 + y_M^2)^(1/2) - 4*L_thigh*k_swLeg*m_M*m_swLeg*theta*sin(theta)*(x_M^2 + y_M^2)^(1/2) + 4*L_thigh*k_swLeg*m_M*m_swLeg*theta0*sin(theta)*(x_M^2 + y_M^2)^(1/2) - 8*L_thigh*k_swLeg*m_M*m_swFoot*theta*sin(theta)*(x_M^2 + y_M^2)^(1/2) + 8*L_thigh*k_swLeg*m_M*m_swFoot*theta0*sin(theta)*(x_M^2 + y_M^2)^(1/2) - 8*L_thigh*k_swLeg*m_swLeg*m_swFoot*theta*sin(theta)*(x_M^2 + y_M^2)^(1/2) + 8*L_thigh*k_swLeg*m_swLeg*m_swFoot*theta0*sin(theta)*(x_M^2 + y_M^2)^(1/2) + 4*L_thigh*dtheta^2*m_swLeg^2*m_swFoot*r^2*cos(theta)*(x_M^2 + y_M^2)^(1/2) + 4*L_thigh^2*dtheta^2*m_swLeg^2*m_swFoot*r*cos(theta)*(x_M^2 + y_M^2)^(1/2) + 4*I_swLeg*L_thigh*dtheta^2*m_M*m_swLeg*cos(theta)*(x_M^2 + y_M^2)^(1/2) + 4*I_swFoot*L_thigh*dtheta^2*m_M*m_swLeg*cos(theta)*(x_M^2 + y_M^2)^(1/2) + 4*I_swLeg*L_thigh*dtheta^2*m_swLeg*m_swFoot*cos(theta)*(x_M^2 + y_M^2)^(1/2) + 4*I_swFoot*L_thigh*dtheta^2*m_swLeg*m_swFoot*cos(theta)*(x_M^2 + y_M^2)^(1/2) - 8*k_swLeg*m_M*m_swFoot*r*theta*sin(theta)*(x_M^2 + y_M^2)^(1/2) + 8*k_swLeg*m_M*m_swFoot*r*theta0*sin(theta)*(x_M^2 + y_M^2)^(1/2) - 8*k_swLeg*m_swLeg*m_swFoot*r*theta*sin(theta)*(x_M^2 + y_M^2)^(1/2) + 8*k_swLeg*m_swLeg*m_swFoot*r*theta0*sin(theta)*(x_M^2 + y_M^2)^(1/2) - 16*L_thigh*k_swFoot*m_M*m_swFoot*r*r0*cos(theta)*(x_M^2 + y_M^2)^(1/2) - 8*L_thigh*k_swFoot*m_swLeg*m_swFoot*r*r0*cos(theta)*(x_M^2 + y_M^2)^(1/2) - 8*L0_ss*L_thigh*k0_ss*m_swLeg*m_swFoot*r*x_M*cos(theta)^2 - 4*L0_ss*L_thigh*k0_ss*m_swLeg*m_swFoot*r*y_M*sin(2*theta) - 4*L_thigh^2*dr*dtheta*m_M*m_swLeg*m_swFoot*sin(theta)*(x_M^2 + y_M^2)^(1/2) - 8*L_thigh*dr*dtheta*m_swLeg^2*m_swFoot*r*sin(theta)*(x_M^2 + y_M^2)^(1/2) + 8*L_thigh*k0_ss*m_swLeg*m_swFoot*r*x_M*cos(theta)^2*(x_M^2 + y_M^2)^(1/2) + 4*L_thigh*k0_ss*m_swLeg*m_swFoot*r*y_M*sin(2*theta)*(x_M^2 + y_M^2)^(1/2) + 4*L_thigh*dtheta^2*m_M*m_swLeg*m_swFoot*r^2*cos(theta)*(x_M^2 + y_M^2)^(1/2) + 8*L_thigh^2*dtheta^2*m_M*m_swLeg*m_swFoot*r*cos(theta)*(x_M^2 + y_M^2)^(1/2) - 8*L_thigh*dr*dtheta*m_M*m_swLeg*m_swFoot*r*sin(theta)*(x_M^2 + y_M^2)^(1/2)))/(2*(x_M^2 + y_M^2)^(1/2)*(m_M + m_swLeg)*(4*I_swLeg*m_M + 4*I_swFoot*m_M + 4*I_swLeg*m_swLeg + 4*I_swLeg*m_swFoot + 4*I_swFoot*m_swLeg + 4*I_swFoot*m_swFoot + 4*m_M*m_swFoot*r^2 + 4*m_swLeg*m_swFoot*r^2 + L_thigh^2*m_M*m_swLeg + 4*L_thigh^2*m_M*m_swFoot + L_thigh^2*m_swLeg*m_swFoot + 8*L_thigh*m_M*m_swFoot*r + 4*L_thigh*m_swLeg*m_swFoot*r))];
            
            % Regularitazation terms
            eps_ss = 1e-7;
            eps_1 = eps_ss/abs(det(A_ss));
            eps_2 = eps_ss/abs(det(A_ss));
            eps_3 = eps_ss/abs(det(A_ss));
            
            E_ss = [
                1/(eps_1 + 1),             0,             0;
                0, 1/(eps_2 + 1),             0;
                0,             0, 1/(eps_3 + 1)];
            
            % U_ss = (A_ss^-1)*K_ss;
            U_ss = E_ss*(A_ss^-1)*K_ss;
            
            det_A_ss = det(A_ss);
            
            u1 = U_ss(1);
            u2 = U_ss(2);
            u3 = U_ss(3);
            
        else
            U_ss = [0;0;0];
            ref_output_ss = [-1; -1; -1];
        end
        %%%%%%%%%%%%%%%%%%%%%%%%%%%%%%%%%%%%%%%%%%%%%%%%%%%%%%%%%%%%%%%%%%
        
        M = [
            m_M + m_swLeg + m_swFoot,                                                                    0,                                 -(sin(theta)*(L_thigh*m_swLeg + 2*L_thigh*m_swFoot + 2*m_swFoot*r))/2, m_swFoot*cos(theta);
            0,                                             m_M + m_swLeg + m_swFoot,                                  (cos(theta)*(L_thigh*m_swLeg + 2*L_thigh*m_swFoot + 2*m_swFoot*r))/2, m_swFoot*sin(theta);
            -(sin(theta)*(L_thigh*m_swLeg + 2*L_thigh*m_swFoot + 2*m_swFoot*r))/2, (cos(theta)*(L_thigh*m_swLeg + 2*L_thigh*m_swFoot + 2*m_swFoot*r))/2, I_swLeg + I_swFoot + (L_thigh^2*m_swLeg)/4 + L_thigh^2*m_swFoot + m_swFoot*r^2 + 2*L_thigh*m_swFoot*r,                   0;
            m_swFoot*cos(theta),                                                  m_swFoot*sin(theta),                                                                                                     0,            m_swFoot;];
        
        H = [
            k0_ss*x_M - 2*dr*dtheta*m_swFoot*sin(theta) - (L_thigh*dtheta^2*m_swLeg*cos(theta))/2 - L_thigh*dtheta^2*m_swFoot*cos(theta) - dtheta^2*m_swFoot*r*cos(theta) - (L0_ss*k0_ss*x_M)/(x_M^2 + y_M^2)^(1/2);
            gravi*m_M + gravi*m_swLeg + gravi*m_swFoot + k0_ss*y_M + 2*dr*dtheta*m_swFoot*cos(theta) - (L_thigh*dtheta^2*m_swLeg*sin(theta))/2 - L_thigh*dtheta^2*m_swFoot*sin(theta) - dtheta^2*m_swFoot*r*sin(theta) - (L0_ss*k0_ss*y_M)/(x_M^2 + y_M^2)^(1/2);
            k_swLeg*theta - k_swLeg*theta0 + 2*dr*dtheta*m_swFoot*r + (L_thigh*gravi*m_swLeg*cos(theta))/2 + L_thigh*gravi*m_swFoot*cos(theta) + gravi*m_swFoot*r*cos(theta) + 2*L_thigh*dr*dtheta*m_swFoot;
            k_swFoot*r - k_swFoot*r0 - dtheta^2*m_swFoot*r + gravi*m_swFoot*sin(theta) - L_thigh*dtheta^2*m_swFoot];
        
        S = [
            -(x_M*(L0_ss - (x_M^2 + y_M^2)^(1/2)))/(x_M^2 + y_M^2)^(1/2),              0,      0;
            -(y_M*(L0_ss - (x_M^2 + y_M^2)^(1/2)))/(x_M^2 + y_M^2)^(1/2),              0,      0;
            0, theta - theta0,      0;
            0,              0, r - r0;];
        
        % U_ss = [0; 0; 0];
        % U_ss = U_ss - [0; U_ss(2); U_ss(3)]; % swing foot goes ahead of the desired trajectory. Testing if it is because of the inputs
        ddq_ss = (M^-1)*(-H - S*U_ss);       
        
        ddx_M = ddq_ss(1);
        ddy_M = ddq_ss(2);
        ddtheta = ddq_ss(3);
        ddr = ddq_ss(4);
        
        ddx_CoM_des = -(L_thigh*ddtheta*m_swLeg*sin(theta) - 2*ddx_M*m_swLeg - 2*ddx_M*m_swFoot - 2*ddr*m_swFoot*cos(theta) - 2*ddx_M*m_M + 2*L_thigh*ddtheta*m_swFoot*sin(theta) + 4*dr*dtheta*m_swFoot*sin(theta) + 2*ddtheta*m_swFoot*r*sin(theta) + L_thigh*dtheta^2*m_swLeg*cos(theta) + 2*L_thigh*dtheta^2*m_swFoot*cos(theta) + 2*dtheta^2*m_swFoot*r*cos(theta))/(2*(m_M + m_swLeg + m_swFoot));
        ddy_CoM_des = (2*ddy_M*m_M + 2*ddy_M*m_swLeg + 2*ddy_M*m_swFoot + 2*ddr*m_swFoot*sin(theta) + L_thigh*ddtheta*m_swLeg*cos(theta) + 2*L_thigh*ddtheta*m_swFoot*cos(theta) + 4*dr*dtheta*m_swFoot*cos(theta) + 2*ddtheta*m_swFoot*r*cos(theta) - L_thigh*dtheta^2*m_swLeg*sin(theta) - 2*L_thigh*dtheta^2*m_swFoot*sin(theta) - 2*dtheta^2*m_swFoot*r*sin(theta))/(2*(m_M + m_swLeg + m_swFoot));
        ddx_sw_des = ddx_M - dtheta*(dr*sin(theta) + dtheta*cos(theta)*(L_thigh + r)) + ddr*cos(theta) - dr*dtheta*sin(theta) - ddtheta*sin(theta)*(L_thigh + r);
        ddy_sw_des = ddy_M + dtheta*(dr*cos(theta) - dtheta*sin(theta)*(L_thigh + r)) + ddr*sin(theta) + dr*dtheta*cos(theta) + ddtheta*cos(theta)*(L_thigh + r);
        
        %         ddx_CoM_des = 0;
        %         ddy_CoM_des = 0;
        %         ddx_sw_des = 0;
        %         ddy_sw_des = 0;
    else
        
        ddx_CoM_des = 0;
        ddy_CoM_des = 0;
        ddx_sw_des = 0;
        ddy_sw_des = 0;
    end
    
else
    % if the system is in DS
    foot_prev = flag(3) - flag(2);
    
    if t_curr_step <= time_ds(end)
        
        %%%%%% V-SLIP-SL SS Phase Controller %%%%%%%%%%%%%%%%%%%%%%%%%%%%%
        % x_CoM = CoM(1) - flag(2); % check this, this might not be a good choice!
        x_CoM = CoM(1) - flag(2); % check this, this might not be a good choice!
        y_CoM = CoM(2);
        dx_CoM = CoM(3);
        dy_CoM = CoM(4);
        
        if x_CoM_star_ds(1) <= x_CoM && x_CoM <= x_CoM_star_ds(end)
            
            % interpolation
            y_CoM_star = interp1(x_CoM_star_ds, ref_star_ds(:,2), x_CoM);
            dx_CoM_star = interp1(x_CoM_star_ds, ref_star_ds(:,3), x_CoM);
            
            del_y_CoM_star = interp1(x_CoM_star_ds, ref_star_ds(:,4), x_CoM);
            del_dx_CoM_star = interp1(x_CoM_star_ds, ref_star_ds(:,5), x_CoM);
            
            del2_y_CoM_star = interp1(x_CoM_star_ds, ref_star_ds(:,6), x_CoM);
            
            ref_output_ds = [y_CoM_star; dx_CoM_star];
            
            A_ds = [
                ((y_CoM - del_y_CoM_star*x_CoM)*(L0_ds - (x_CoM^2 + y_CoM^2)^(1/2)))/((x_CoM^2 + y_CoM^2)^(1/2)*(m_M + m_swLeg + m_swFoot)), (y_CoM*(L0_ds/(y_CoM^2 + (foot_prev - x_CoM)^2)^(1/2) - 1))/(m_M + m_swLeg + m_swFoot) + (del_y_CoM_star*(foot_prev - x_CoM)*(L0_ds/(y_CoM^2 + (foot_prev - x_CoM)^2)^(1/2) - 1))/(m_M + m_swLeg + m_swFoot)
                (x_CoM*(L0_ds/(x_CoM^2 + y_CoM^2)^(1/2) - 1))/(m_M + m_swLeg + m_swFoot),                                                                                                        -((foot_prev - x_CoM)*(L0_ds/(y_CoM^2 + (foot_prev - x_CoM)^2)^(1/2) - 1))/(m_M + m_swLeg + m_swFoot)];
            
            K_ds = [
                del2_y_CoM_star*dx_CoM^2 - K_p_ds*(y_CoM - y_CoM_star) - K_d_ds*(dy_CoM - del_y_CoM_star*dx_CoM) - (k0_ds*y_CoM*(L0_ds/(x_CoM^2 + y_CoM^2)^(1/2) - 1) - gravi*(m_M + m_swLeg + m_swFoot) + k0_ds*y_CoM*(L0_ds/(y_CoM^2 + (foot_prev - x_CoM)^2)^(1/2) - 1))/(m_M + m_swLeg + m_swFoot) - (del_y_CoM_star*(k0_ds*(foot_prev - x_CoM)*(L0_ds/(y_CoM^2 + (foot_prev - x_CoM)^2)^(1/2) - 1) - k0_ds*x_CoM*(L0_ds/(x_CoM^2 + y_CoM^2)^(1/2) - 1)))/(m_M + m_swLeg + m_swFoot);
                del_dx_CoM_star*dx_CoM - K_v_ds*(dx_CoM - dx_CoM_star) + (k0_ds*(foot_prev - x_CoM)*(L0_ds/(y_CoM^2 + (foot_prev - x_CoM)^2)^(1/2) - 1) - k0_ds*x_CoM*(L0_ds/(x_CoM^2 + y_CoM^2)^(1/2) - 1))/(m_M + m_swLeg + m_swFoot)];
            
            % regularization terms
            %         eps_ds = 5e-5;
            %         eps_4 = eps_ds/det(A_ds);
            %         eps_5 = eps_ds/det(A_ds);
            %
            %         E_ds = [1/(eps_4 + 1), 0; 0, 1/(eps_5 + 1)];
            
            %         U_ds = E_ds*(A_ds^-1)*K_ds;
            
            det_A_ds = det(A_ds);

            %u4 = U_ds(1);
            %u5 = U_ds(2);
            
            if abs(det_A_ds) >= 4e-9
                U_ds = (A_ds^-1)*K_ds;
                u4 = U_ds(1);
                u5 = U_ds(2);
                
                % u4 = 0;
                %u5 = 0;
            else
                u4 = 0;
                u5 = 0;
            end
        end
        %%%%%%%%%%%%%%%%%%%%%%%%%%%%%%%%%%%%%%%%%%%%%%%%%%%%%%%%%%%%%%%%%%
        
        % temporary!!!
        % foot = foot;
        % foot_prev = foot - 0.25;
        
        L1 = sqrt((x_CoM - foot)^2 + y_CoM^2); % length of the new stance leg
        L2 = sqrt((x_CoM - foot_prev)^2 + y_CoM^2); % length of the old stance leg
        
        Fs1 = (k0_ds + u4) * ((L0_ds/L1) - 1) * [x_CoM - foot; y_CoM]; % Spring force of the new stance leg
        Fs2 = (k0_ds + u5) * ((L0_ds/L2 )- 1) * [x_CoM - foot_prev; y_CoM]; % Spring force of the old stance leg
        F = Fs1 + Fs2; % spring force matrix
        
        ddq_ds = [
            (F(1))/(m_M + m_swLeg + m_swFoot);
            (F(2) - (m_M + m_swLeg + m_swFoot)*gravi)/(m_M + m_swLeg + m_swFoot)];
        
        ddx_CoM_des = ddq_ds(1);
        ddy_CoM_des = ddq_ds(2);
        ddx_sw_des = 0;
        ddy_sw_des = 0;
    else
        ddx_CoM_des = 0;
        ddy_CoM_des = 0;
        ddx_sw_des = 0;
        ddy_sw_des = 0;
    end
end

% SLIP-SL desired accelerations
% ddx_CoM_des = 0;
% ddy_CoM_des = 0;
% ddx_sw_des = 0;
% ddy_sw_des = 0;

input_varStiff = [u1; u2; u3; u4; u5];

%% outputs
des_traj = [
    ddx_CoM_des; ddy_CoM_des; ddx_sw_des; ddy_sw_des;
    dx_CoM_des;  dy_CoM_des;  dx_sw_des;  dy_sw_des;
    x_CoM_des;   y_CoM_des;   x_sw_des;   y_sw_des];

flag_des = flag_des;

%% finding the desired joint angles
[des_th, decoder_time_elapsed] = calc_desJointAngles(X, des_traj, flag, param, flag_des);
